simulink model "ADU_Integration_R2014a_simulation"  (R2014a)
settings: Solver=FixedStepDiscrete  StartTime=285  StopTime=300  FixedStep=0.01  RelTol=1e-3
PostLoadFcn:
  | , if any(exist('dsrtsu_mdlpostloadfcn', 'file') == [2, 3, 6]), try dsrtsu_mdlpostloadfcn('Execute', bdroot); catch fprintf('Error in PostLoadFcn (dsrtsu_mdlpostloadfcn) for model "%s":\n %s\n', bdroot, lasterr); end, end,
InitFcn:
  | load 'data/chi2_dat';
  | load 'data/Line_struct';
  | load 'data/innerLNM_1';
  | load 'data/middleLNM_2';
  | load 'data/outerLNM_1';
  | load 'data/landmarks_patac_schimmel_ccw';
  | load 'data/patac_navi_array';
  | load 'data/sensor';
  | load 'data/map_struct';
  | addpath map_src
  | Integration_Parameter;
  | load 'TestData_001';
values from neighbouring files (symbols this model uses):
  TestData_001 =     [TestData_001.mat]
undefined symbols (not defined in the file or in its folder): chi2_dat, innerLNM_1, landmarks_patac_schimmel_ccw, middleLNM_2, outerLNM_1, patac_navi_array
libraries: simulink x36, rtican x1
(part 13 of 22)

== stateflow chart ADU_Integration_R2014a_simulation/Fusion_Model/Fusion_Block/Side_Fusion/Side_Fusion ==
  state Gtj  = G_cal(xt,yt,xj,yj,P11,P12,P13,P14,P21,P22,P23,P24,... [function]
    P31,P32,P33,P34,P41,P42,P43,P44,R11,R12,R21,R22)
  state Set_Source(data) [function]
    (default) -> (junction 1307)
    (junction 1307) -> (junction 1308) : {
        | DataSource = data;
        | }
  state Tracker_Update [function]
    state Tracker_Filter [function]
      state Measurement_Select [function]
        state Data_Gen [function]
          (default) -> (junction 648)
          (junction 648) -> (junction 650) [order 1] : [j<Measure_Num]
          (junction 656) -> (junction 648) : {
              | j++;
              | }
          (junction 648) -> (junction 661) [order 2] : {
              | j=0;
              | }
          (junction 650) -> (junction 656) : {
              | P_Bulb[j][0]=Ptj[t][j];
              | P_Bulb[j][1]=Measure_Data[j][1]-FusDataInternal[t][1];
              | P_Bulb[j][2]=Measure_Data[j][2]-FusDataInternal[t][3];
              | P_Bulb[j][3]=j;%Used to define the measurement is used
              | }
        state Bulb_Sort [function]
          (default) -> (junction 638) : {
              | P_Bulbtemp0=0;P_Bulbtemp1=0;P_Bulbtemp2=0;
              | LoopFlg=1;
              | }
          (junction 2794) -> (junction 2793) [order 1] : [P_Bulb[j][0]>P_Bulb[j+1][0]]
          (junction 2800) -> (junction 2794) [order 1] : [j<Measure_Num-1]
          (junction 2813) -> (junction 2800) : {LoopFlg=0;}
          (junction 638) -> (junction 639) [order 1] : [LoopFlg==1]
          (junction 639) -> (junction 2813) [order 1] : [Measure_Num>2]
          (junction 2794) -> (junction 2790) [order 2]
          (junction 2793) -> (junction 2791) : {
              | P_Bulbtemp0=P_Bulb[j][0];P_Bulbtemp1=P_Bulb[j][1];
              | P_Bulbtemp2=P_Bulb[j][2];P_Bulbtemp3=P_Bulb[j][3];
              | P_Bulb[j][0]=P_Bulb[j+1][0];P_Bulb[j][1]=P_Bulb[j+1][1];
              | P_Bulb[j][2]=P_Bulb[j+1][2];P_Bulb[j][3]=P_Bulb[j+1][3];
              | P_Bulb[j+1][0]=P_Bulbtemp0;P_Bulb[j+1][1]=P_Bulbtemp1;
              | P_Bulb[j+1][2]=P_Bulbtemp2;P_Bulb[j+1][3]=P_Bulbtemp3;
              | LoopFlg=1;
              | }
          (junction 2817) -> (junction 638) : {
              | j=0;
              | }
          (junction 638) -> (junction 679) [order 2]
          (junction 2790) -> (junction 2800) : {
              | j++;
              | }
          (junction 2800) -> (junction 2802) [order 2]
          (junction 639) -> (junction 2815) [order 2]
          (junction 2815) -> (junction 2805) [order 1] : [Measure_Num>1]
          (junction 2805) -> (junction 2808) [order 1] : [P_Bulb[0][0]>P_Bulb[1][0]]
          (junction 2815) -> (junction 2817) [order 2] : {
              | LoopFlg=0;
              | }
          (junction 2805) -> (junction 675) [order 2] : {
              | LoopFlg=0;
              | }
          (junction 2808) -> (junction 2809) : {
              | P_Bulbtemp0=P_Bulb[0][0];P_Bulbtemp1=P_Bulb[0][1];
              | P_Bulbtemp2=P_Bulb[0][2];P_Bulbtemp3=P_Bulb[0][3];
              | P_Bulb[0][0]=P_Bulb[1][0];P_Bulb[0][1]=P_Bulb[1][1];
              | P_Bulb[0][2]=P_Bulb[1][2];P_Bulb[0][3]=P_Bulb[1][3];
              | P_Bulb[1][0]=P_Bulbtemp0;P_Bulb[1][1]=P_Bulbtemp1;
              | P_Bulb[1][2]=P_Bulbtemp2;P_Bulb[1][3]=P_Bulbtemp3;
              | LoopFlg=0;
              | }
          (junction 2791) -> (junction 2790)
          (junction 675) -> (junction 2817)
          (junction 2802) -> (junction 2809)
          (junction 2809) -> (junction 675)
        state Measure_Select [function]
          note: this part is select the 6  highest possible measurement to update
              | Tracker, and make sure if possible lower than 15%, think the date
              | as unused.
          (default) -> (junction 682) : {mk=0;}
          (junction 682) -> (junction 2830) [order 1] : [Measure_Num>2]
          (junction 2830) -> (junction 2829) [order 1] : [k<3]
          (junction 2829) -> (junction 2825) [order 1] : [P_Bulb[Measure_Num-1-k][0]>Poss_Threshold_used]
          (junction 2826) -> (junction 2830) : {
              | k++;
              | }
          (junction 682) -> (junction 715) [order 2]
          (junction 2830) -> (junction 2832) [order 2]
          (junction 2829) -> (junction 2826) [order 2]
          (junction 2825) -> (junction 2821) : {
              | SelectMea[k][0]=P_Bulb[Measure_Num-1-k][0];
              | SelectMea[k][1]=P_Bulb[Measure_Num-1-k][1];
              | SelectMea[k][2]=P_Bulb[Measure_Num-1-k][2];
              | Measure_Data[P_Bulb[Measure_Num-1-k][3]][4]=1;%Means that the measurement is used
              | mk++;
              | }
          (junction 2832) -> (junction 715)
          (junction 2821) -> (junction 2826)
          (junction 715) -> (junction 2835) : {
              | k=0;
              | }
          (junction 2837) -> (junction 2849) [order 1] : [k<2]
          (junction 2835) -> (junction 2837) [order 1] : [Measure_Num==2]
          (junction 2849) -> (junction 2847) [order 1] : [P_Bulb[Measure_Num-1-k][0]>Poss_Threshold_used]
          (junction 2844) -> (junction 2837) : {
              | k++;
              | }
          (junction 2849) -> (junction 2844) [order 2]
          (junction 2835) -> (junction 2853) [order 2]
          (junction 2837) -> (junction 2850) [order 2]
          (junction 2847) -> (junction 2846) : {
              | SelectMea[k][0]=P_Bulb[Measure_Num-1-k][0];
              | SelectMea[k][1]=P_Bulb[Measure_Num-1-k][1];
              | SelectMea[k][2]=P_Bulb[Measure_Num-1-k][2];
              | Measure_Data[P_Bulb[Measure_Num-1-k][3]][4]=1;%Means that the measurement is used
              | mk++;
              | }
          (junction 2850) -> (junction 2853)
          (junction 2846) -> (junction 2844)
          (junction 2853) -> (junction 2871) : {
              | k=0;
              | }
          (junction 2867) -> (junction 2861) [order 1] : [k<1]
          (junction 2871) -> (junction 2867) [order 1] : [Measure_Num==1]
          (junction 2861) -> (junction 2872) [order 1] : [P_Bulb[Measure_Num-1-k][0]>Poss_Threshold_used]
          (junction 2868) -> (junction 2867) : {
              | k++;
              | }
          (junction 2861) -> (junction 2868) [order 2]
          (junction 2871) -> (junction 2873) [order 2]
          (junction 2867) -> (junction 2865) [order 2]
          (junction 2872) -> (junction 2866) : {
              | SelectMea[k][0]=P_Bulb[Measure_Num-1-k][0];
              | SelectMea[k][1]=P_Bulb[Measure_Num-1-k][1];
              | SelectMea[k][2]=P_Bulb[Measure_Num-1-k][2];
              | Measure_Data[P_Bulb[Measure_Num-1-k][3]][4]=1;%Means that the measurement is used
              | mk++;
              | }
          (junction 2865) -> (junction 2873)
          (junction 2866) -> (junction 2868)
          (junction 2873) -> (junction 2875) : {
              | k=0;
              | }
          (junction 2875) -> (junction 3173)
          (junction 3173) -> (junction 3175) [order 1] : [mk==1]%means that the tracker
              | %only has one measurement
          (junction 3175) -> (junction 3177) [order 1] : [OneMeasureFlg[P_Bulb[Measure_Num-1-k][3]]==1]
              | %Means that the measurement has used for another tracker
              | %and this tracker only has one measurement
          (junction 3173) -> (junction 3184) [order 2]
          (junction 3175) -> (junction 3181) [order 2] : {
              | OneMeasureFlg[P_Bulb[Measure_Num-1-k][3]]=1;
              | %Means that this measurement has used for another track and the track
              | %only has one measurement
              | }
          (junction 3177) -> (junction 3179) : {
              | mk=0;%Means that no measurement here
              | }
          (junction 3181) -> (junction 3184)
          (junction 3179) -> (junction 3181)
          (junction 3184) -> (junction 3187)
          (junction 3187) -> (junction 3280) [order 1] : [j<Measure_Num]
          (junction 3280) -> (junction 3282) [order 1] : [P_Bulb[j][0]>Poss_Threshold_unused]
          (junction 3286) -> (junction 3187) : {
              | j++;
              | }
          (junction 3187) -> (junction 3290) [order 2] : {
              | j=0;
              | }
          (junction 3280) -> (junction 3286) [order 2]
          (junction 3282) -> (junction 3284) : {
              | Measure_Data[P_Bulb[j][3]][4]=1;
              | }
          (junction 3284) -> (junction 3286)
        (default) -> (junction 630) : {
            | LoopFlg=1;SelectMea=0;
            | %This Step is to select measurements to update the tracker, the measurement used
            | }
        (junction 630) -> (junction 635) : {
            | Data_Gen();
            | Bulb_Sort();
            | Measure_Select();
            | }
      state Update [function]
        state [RangeX,VelX,RangeY,VelY,P11,P12,P13,P14,P21,P22,P23,P24,P31,P32,P33,P34,P41,P42,P43,... [function]
          P44] = Update(Pre_x,Pre_vx,Pre_y,Pre_vy,pre_p11,pre_p12,pre_p13,pre_p14,pre_p21,pre_p22,...
          pre_p23,pre_p24,pre_p31,pre_p32,pre_p33,pre_p34,pre_p41,pre_p42,pre_p43,pre_p44,mk,m00,...
          m01,m2,m10,m11,m12,m20,m21,m22,Pt0)
        (default) -> (junction 718)
        (junction 718) -> (junction 768) [order 1] : [mk>0]%Exist Measurement can update Tracker
        (junction 718) -> (junction 719) [order 2] : {
            | UpdateTrackFlag[t]=0;%Could not find measurement to update tracker
            | FusDataInternal_temp[t][0]=FusDataInternal[t][0];FusDataInternal_temp[t][1]=FusDataInternal[t][1];
            | FusDataInternal_temp[t][2]=FusDataInternal[t][2];FusDataInternal_temp[t][3]=FusDataInternal[t][3];
            | FusDataInternal_temp[t][4]=FusDataInternal[t][4];FusDataInternal_temp[t][5]=FusDataInternal[t][5];
            | FusDataInternal_temp[t][6]=FusDataInternal[t][6];FusDataInternal_temp[t][7]=FusDataInternal[t][7];
            | FusDataInternal_temp[t][8]=FusDataInternal[t][8];FusDataInternal_temp[t][9]=FusDataInternal[t][9];
            | FusDataInternal_temp[t][10]=FusDataInternal[t][10];FusDataInternal_temp[t][11]=FusDataInternal[t][11];
            | FusDataInternal_temp[t][12]=FusDataInternal[t][12];FusDataInternal_temp[t][13]=FusDataInternal[t][13];
            | FusDataInternal_temp[t][14]=FusDataInternal[t][14];FusDataInternal_temp[t][15]=FusDataInternal[t][15];
            | FusDataInternal_temp[t][16]=FusDataInternal[t][16];FusDataInternal_temp[t][17]=FusDataInternal[t][17];
            | FusDataInternal_temp[t][18]=FusDataInternal[t][18];FusDataInternal_temp[t][19]=FusDataInternal[t][19];
            | FusDataInternal_temp[t][20]=FusDataInternal[t][20];FusDataInternal_temp[t][21]=FusDataInternal[t][21];
            | FusDataInternal_temp[t][22]=FusDataInternal[t][22];
            | FusDataInternal_temp[t][23]=FusDataInternal[t][23];FusDataInternal_temp[t][24]=FusDataInternal[t][24];
            | }
        (junction 768) -> (junction 771) : {
            | UpdateTrackFlag[t]=1;
            | [FusDataInternal_temp[t][1],FusDataInternal_temp[t][2],FusDataInternal_temp[t][3],FusDataInternal_temp[t][4],...
            | FusDataInternal_temp[t][7],FusDataInternal_temp[t][8],FusDataInternal_temp[t][9],FusDataInternal_temp[t][10],...
            | FusDataInternal_temp[t][11],FusDataInternal_temp[t][12],FusDataInternal_temp[t][13],FusDataInternal_temp[t][14],...
            | FusDataInternal_temp[t][15],FusDataInternal_temp[t][16],FusDataInternal_temp[t][17],FusDataInternal_temp[t][18],...
            | FusDataInternal_temp[t][19],FusDataInternal_temp[t][20],FusDataInternal_temp[t][21],FusDataInternal_temp[t][22]]=Update(FusDataInternal[t][1],...
            | FusDataInternal[t][2],FusDataInternal[t][3],FusDataInternal[t][4],FusDataInternal[t][7],FusDataInternal[t][8],FusDataInternal[t][9],...
            | FusDataInternal[t][10],FusDataInternal[t][11],FusDataInternal[t][12],FusDataInternal[t][13],FusDataInternal[t][14],FusDataInternal[t][15],...
            | FusDataInternal[t][16],FusDataInternal[t][17],FusDataInternal[t][18],FusDataInternal[t][19],FusDataInternal[t][20],FusDataInternal[t][21],...
            | FusDataInternal[t][22],mk,SelectMea[0][0],SelectMea[0][1],SelectMea[0][2],SelectMea[1][0],SelectMea[1][1],SelectMea[1][2],SelectMea[2][0],...
            | SelectMea[2][1],SelectMea[2][2],(1-Ptsum[t]));
            | FusDataInternal_temp[t][0]=FusDataInternal[t][0];FusDataInternal_temp[t][5]=FusDataInternal[t][5];FusDataInternal_temp[t][6]=FusDataInternal[t][6];
            | FusDataInternal_temp[t][23]=FusDataInternal[t][23];FusDataInternal_temp[t][24]=FusDataInternal[t][24];
            | }
        (junction 771) -> (junction 719)
        (junction 719) -> (junction 825)
      (default) -> (junction 626)
      (junction 626) -> (junction 627) : {
          | Measurement_Select();
          | Update();
          | }
    (default) -> (junction 607)
    (junction 607) -> (junction 608) [order 1] : [t<Num_Trg]
    (junction 610) -> (junction 607) : {
        | t++;
        | }
    (junction 607) -> (junction 613) [order 2] : {
        | t=0;
        | }
    (junction 608) -> (junction 610) : {
        | Tracker_Filter();
        | }
  state Set_Time(data) [function]
    (default) -> (junction 1301)
    (junction 1301) -> (junction 1302) : {
        | Sensor_sampleTime = data;
        | }
  state FusDataIni [function]
    (default) -> (junction 206)
    (junction 206) -> (junction 207) : {
        | %deltaT=0;
        | deltaT=Sensor_sampleTime-LastCalTime;
        | TrackCounter=0;c=0;Num_Out=0;
        | Gtj=0;Ptj=0;Measure_Data=0;Gtsum=0;Gsumj=0;Ptsum=0;Psumj=0;
        | Measure_Data=0;Measure_Num=0;Tracker_Num=0;k=0;n=0;t=0;j=0;
        | SideFusOut=0;Returns=0;Num_Returns=0;OneMeasureFlg=0;
        | FusDataInternal=0;Pt0=0;P_Bulb=0;UpdateTrackFlag=0;SelectMea=0;
        | }
    (junction 207) -> (junction 208)
  state FusTrackPredict [function]
    state [RangeX,VelX,RangeY,VelY,P11,P12,P13,P14,P21,P22,P23,P24,P31,P32,P33,P34,P41,P42,P43,... [function]
      P44] = Forecast(Pre_x,Pre_vx,Pre_y,Pre_vy,deltaT,pre_p11,pre_p12,pre_p13,pre_p14,pre_p21,...
      pre_p22,pre_p23,pre_p24,pre_p31,pre_p32,pre_p33,pre_p34,pre_p41,pre_p42,pre_p43,pre_p44)
    (default) -> (junction 330)
    (junction 330) -> (junction 331) [order 1] : [k<Num_Trg]
    (junction 331) -> (junction 332) [order 1] : [FusDataInternal_temp[k][0]!=0]
    (junction 333) -> (junction 330) : {
        | k++;
        | }
    (junction 330) -> (junction 335) [order 2] : {
        | Num_Trg=n;
        | n=0;
        | }
    (junction 331) -> (junction 333) [order 2]
    (junction 332) -> (junction 334) : {
        | [FusDataInternal[n][1],FusDataInternal[n][2],FusDataInternal[n][3],FusDataInternal[n][4],FusDataInternal[n][7],FusDataInternal[n][8],FusDataInternal[n][9],FusDataInternal[n][10],...
        | FusDataInternal[n][11],FusDataInternal[n][12],FusDataInternal[n][13],FusDataInternal[k][14],FusDataInternal[k][15],FusDataInternal[k][16],FusDataInternal[n][17],FusDataInternal[n][18],...
        | FusDataInternal[n][19],FusDataInternal[n][20],FusDataInternal[n][21],FusDataInternal[n][22]]=Forecast(FusDataInternal_temp[k][1],FusDataInternal_temp[k][2],FusDataInternal_temp[k][3],...
        | FusDataInternal_temp[k][4],deltaT,FusDataInternal_temp[k][7],FusDataInternal_temp[k][8],FusDataInternal_temp[k][9],FusDataInternal_temp[k][10],FusDataInternal_temp[k][11],FusDataInternal_temp[k][12],...
        | FusDataInternal_temp[k][13],FusDataInternal_temp[k][14],FusDataInternal_temp[k][15],FusDataInternal_temp[k][16],FusDataInternal_temp[k][17],FusDataInternal_temp[k][18],FusDataInternal_temp[k][19],...
        | FusDataInternal_temp[k][20],FusDataInternal_temp[k][21],FusDataInternal_temp[k][22]);%All fusion targets forecast,after this step, target number in FusDataInternal is the same as last calculation, but forecast with delta time
        | FusDataInternal[n][0]=FusDataInternal_temp[k][0];FusDataInternal[n][5]=FusDataInternal_temp[k][5];FusDataInternal[n][6]=FusDataInternal_temp[k][6];
        | FusDataInternal[n][23]=FusDataInternal_temp[k][23];FusDataInternal[n][24]=FusDataInternal_temp[k][24];
        | n++;
        | }
    (junction 334) -> (junction 333)
  state Tracker_Initial [function]
    state Unused_Return_Gen [function]
      (default) -> (junction 1656) : {
          | Num_Returns=0;
          | }
      (junction 1656) -> (junction 1662) [order 1] : [k<Measure_Num]
      (junction 1662) -> (junction 1664) [order 1] : [Measure_Data[k][4]==0]
      (junction 1670) -> (junction 1656) : {
          | k++;
          | }
      (junction 1656) -> (junction 1674) [order 2] : {
          | k=0;
          | }
      (junction 1662) -> (junction 1670) [order 2]
      (junction 1664) -> (junction 1666) : {
          | Returns[Num_Returns][0]=Measure_Data[k][1];
          | Returns[Num_Returns][1]=Measure_Data[k][2];
          | Returns[Num_Returns][2]=Measure_Data[k][4];
          | Num_Returns++;
          | }
      (junction 1666) -> (junction 1670)
    state LFSRR_Ini [function]
      state LFSRR_Ini_Update [function]
        note: %Recently used in 4/5 logical modle in the initial of radar tracker
        state Ini_FifthTime_LF [function]
          (default) -> (junction 2080) : {
              | RelDeg=0;Min_Distance_IniTrack=9;RelativeDist=0;
              | x_5_predict=3*Ini_Tracker_LFSRR[k][10]-3*Ini_Tracker_LFSRR[k][8]+Ini_Tracker_LFSRR[k][6];%Use three point to predict next point based constant acc
              | y_5_predict=3*Ini_Tracker_LFSRR[k][11]-3*Ini_Tracker_LFSRR[k][9]+Ini_Tracker_LFSRR[k][7];%Use three point to predict next point based constant acc
              | Updatereturn=0;Ini_Tracker_UpdateFlg=0;
              | }
          (junction 2080) -> (junction 2890) [order 1] : [(j<Num_Returns)]
          (junction 2890) -> (junction 2091) [order 1] : [(Returns[j][2]==0)]
          (junction 2892) -> (junction 2080) : {
              | j++;
              | }
          (junction 2091) -> (junction 2108) : {
              | RelativeDist=(x_5_predict-Returns[j][0])*(x_5_predict-Returns[j][0])+(y_5_predict-Returns[j][1])*(y_5_predict-Returns[j][1]);
              | RelDeg=cos_cal(Ini_Tracker_LFSRR[k][8],Ini_Tracker_LFSRR[k][9],...
              | Ini_Tracker_LFSRR[k][10],Ini_Tracker_LFSRR[k][11],Returns[j][0],Returns[j][1]);
              | }
          (junction 2080) -> (junction 2102) [order 2] : {
              | j=0;
              | }
          (junction 2890) -> (junction 2892) [order 2]
          (junction 2108) -> (junction 2987) [order 1] : [(RelativeDist<4)]
          (junction 2987) -> (junction 2990) [order 1] : [(RelativeDist<0.1)]
          (junction 2108) -> (junction 2107) [order 2]
          (junction 2987) -> (junction 2991) [order 2]
          (junction 2990) -> (junction 2973)
          (junction 2991) -> (junction 2973) [order 1] : [(((RelDeg>120) || (RelDeg<60)))]
          (junction 2973) -> (junction 2977) [order 1] : [RelativeDist<Min_Distance_IniTrack]
          (junction 2991) -> (junction 2985) [order 2]
          (junction 2973) -> (junction 2981) [order 2]
          (junction 2977) -> (junction 2979) : {
              | Updatereturn=j;
              | Ini_Tracker_UpdateFlg=1;
              | Min_Distance_IniTrack=RelativeDist;
              | }
          (junction 2981) -> (junction 2985)
          (junction 2979) -> (junction 2981)
          (junction 2985) -> (junction 2107)
          (junction 2107) -> (junction 2892)
          (junction 2102) -> (junction 2104) [order 1] : [Ini_Tracker_UpdateFlg==1]%Means that the tracker k found measurement
          (junction 2102) -> (junction 2094) [order 2] : {
              | %cound not found, and enter 5 searches means that could not found once before, so delete
              | }
          (junction 2104) -> (junction 2100) : {
              | Returns[Updatereturn][2]=1;
              | %Which means that the return is used
              | TrackIni(Returns[Updatereturn][0],Returns[Updatereturn][1]);
              | }
          (junction 2100) -> (junction 2094)
          (junction 2094) -> (junction 2105) : {
              | Updatereturn=0;Ini_Tracker_UpdateFlg=0;
              | }
        state Ini_ForthTime_LF [function]
          (default) -> (junction 2039) : {
              | RelDeg=0;Min_Distance_IniTrack=9;RelativeDist=0;
              | x_4_predict=3*Ini_Tracker_LFSRR[k][8]-3*Ini_Tracker_LFSRR[k][6]+Ini_Tracker_LFSRR[k][4];%Use three point to predict next point based constant acc
              | y_4_predict=3*Ini_Tracker_LFSRR[k][9]-3*Ini_Tracker_LFSRR[k][7]+Ini_Tracker_LFSRR[k][5];%Use three point to predict next point based constant acc
              | Updatereturn=0;Ini_Tracker_UpdateFlg=0;
              | }
          (junction 2039) -> (junction 2885) [order 1] : [(j<Num_Returns)]
          (junction 2885) -> (junction 2047) [order 1] : [(Returns[j][2]==0)]
          (junction 2887) -> (junction 2039) : {
              | j++;
              | }
          (junction 2047) -> (junction 2044) : {
              | RelativeDist=(x_4_predict-Returns[j][0])*(x_4_predict-Returns[j][0])+(y_4_predict-Returns[j][1])*(y_4_predict-Returns[j][1]);
              | RelDeg=cos_cal(Ini_Tracker_LFSRR[k][6],Ini_Tracker_LFSRR[k][7],...
              | Ini_Tracker_LFSRR[k][8],Ini_Tracker_LFSRR[k][9],Returns[j][0],Returns[j][1]);
              | }
          (junction 2039) -> (junction 2053) [order 2] : {
              | j=0;
              | }
          (junction 2885) -> (junction 2887) [order 2]
          (junction 2044) -> (junction 2967) [order 1] : [(RelativeDist<4)]
          (junction 2967) -> (junction 2970) [order 1] : [(RelativeDist<0.1)]
          (junction 2044) -> (junction 2036) [order 2]
          (junction 2967) -> (junction 2971) [order 2]
          (junction 2970) -> (junction 2953)
          (junction 2971) -> (junction 2953) [order 1] : [(((RelDeg>120) || (RelDeg<60)))]
          (junction 2953) -> (junction 2957) [order 1] : [RelativeDist<Min_Distance_IniTrack]
          (junction 2971) -> (junction 2965) [order 2]
          (junction 2953) -> (junction 2961) [order 2]
          (junction 2957) -> (junction 2959) : {
              | Updatereturn=j;
              | Ini_Tracker_UpdateFlg=1;
              | Min_Distance_IniTrack=RelativeDist;
              | }
          (junction 2036) -> (junction 2887)
          (junction 2965) -> (junction 2036)
          (junction 2961) -> (junction 2965)
          (junction 2959) -> (junction 2961)
          (junction 2053) -> (junction 2052) [order 1] : [Ini_Tracker_UpdateFlg==1]%Means that the tracker k found measurement
          (junction 2052) -> (junction 2064) [order 1] : [Ini_Tracker_LFSRR[k][3]==3]%Has found measurement 4 times and begin ini
          (junction 2053) -> (junction 2071) [order 2]
          (junction 2052) -> (junction 2049) [order 2] : {
              | Returns[Updatereturn][2]=1;%Which means that the return is used
              | Ini_Tracker_LFSRR_New[Num_Ini_Tracker_LFSRR_New][0]=Returns[Updatereturn][0];
              | Ini_Tracker_LFSRR_New[Num_Ini_Tracker_LFSRR_New][1]=Returns[Updatereturn][1];
              | Ini_Tracker_LFSRR_New[Num_Ini_Tracker_LFSRR_New][2]=4;%Tracker counter
              | Ini_Tracker_LFSRR_New[Num_Ini_Tracker_LFSRR_New][3]=3;%Association counter
              | Ini_Tracker_LFSRR_New[Num_Ini_Tracker_LFSRR_New][4]=Ini_Tracker_LFSRR[k][4];
              | Ini_Tracker_LFSRR_New[Num_Ini_Tracker_LFSRR_New][5]=Ini_Tracker_LFSRR[k][5];
              | Ini_Tracker_LFSRR_New[Num_Ini_Tracker_LFSRR_New][6]=Ini_Tracker_LFSRR[k][6];
              | Ini_Tracker_LFSRR_New[Num_Ini_Tracker_LFSRR_New][7]=Ini_Tracker_LFSRR[k][7];
              | Ini_Tracker_LFSRR_New[Num_Ini_Tracker_LFSRR_New][8]=Ini_Tracker_LFSRR[k][8];
              | Ini_Tracker_LFSRR_New[Num_Ini_Tracker_LFSRR_New][9]=Ini_Tracker_LFSRR[k][9];
              | Ini_Tracker_LFSRR_New[Num_Ini_Tracker_LFSRR_New][10]=Returns[Updatereturn][0];
              | Ini_Tracker_LFSRR_New[Num_Ini_Tracker_LFSRR_New][11]=Returns[Updatereturn][1];
              | Num_Ini_Tracker_LFSRR_New++;
              | }
          (junction 2064) -> (junction 2068) : {
              | Returns[Updatereturn][2]=1;
              | %Which means that the return is used
              | TrackIni(Returns[Updatereturn][0],Returns[Updatereturn][1]);
              | }
          (junction 2071) -> (junction 2073) [order 1] : [Ini_Tracker_LFSRR[k][3]==3]
              | %Has found measurement 3 times before
          (junction 2073) -> (junction 2075) : {
              | Ini_Tracker_LFSRR_New[Num_Ini_Tracker_LFSRR_New][0]=x_4_predict;
              | Ini_Tracker_LFSRR_New[Num_Ini_Tracker_LFSRR_New][1]=y_4_predict;
              | Ini_Tracker_LFSRR_New[Num_Ini_Tracker_LFSRR_New][2]=4;%Tracker counter
              | Ini_Tracker_LFSRR_New[Num_Ini_Tracker_LFSRR_New][3]=3;%Association counter
              | Ini_Tracker_LFSRR_New[Num_Ini_Tracker_LFSRR_New][4]=Ini_Tracker_LFSRR[k][4];
              | Ini_Tracker_LFSRR_New[Num_Ini_Tracker_LFSRR_New][5]=Ini_Tracker_LFSRR[k][5];
              | Ini_Tracker_LFSRR_New[Num_Ini_Tracker_LFSRR_New][6]=Ini_Tracker_LFSRR[k][6];
              | Ini_Tracker_LFSRR_New[Num_Ini_Tracker_LFSRR_New][7]=Ini_Tracker_LFSRR[k][7];
              | Ini_Tracker_LFSRR_New[Num_Ini_Tracker_LFSRR_New][8]=Ini_Tracker_LFSRR[k][8];
              | Ini_Tracker_LFSRR_New[Num_Ini_Tracker_LFSRR_New][9]=Ini_Tracker_LFSRR[k][9];
              | Ini_Tracker_LFSRR_New[Num_Ini_Tracker_LFSRR_New][10]=x_4_predict;
              | Ini_Tracker_LFSRR_New[Num_Ini_Tracker_LFSRR_New][11]=y_4_predict;
              | Num_Ini_Tracker_LFSRR_New++;
              | }
          (junction 2071) -> (junction 2054) [order 2] : {
              | %Cound not found measurement twice,
              | % So not transfer tracker k to new list
              | }
          (junction 2075) -> (junction 2054)
          (junction 2049) -> (junction 2075)
          (junction 2068) -> (junction 2049)
          (junction 2054) -> (junction 2057) : {
              | Updatereturn=0;Ini_Tracker_UpdateFlg=0;
              | }
        state Ini_ThridTime_LF [function]
          (default) -> (junction 1976) : {
              | RelDeg=0;Min_Distance_IniTrack=9;RelativeDist=0;
              | x_3_predict=2*Ini_Tracker_LFSRR[k][6]-Ini_Tracker_LFSRR[k][4];%Use two point to predict next point based constant velocity
              | y_3_predict=2*Ini_Tracker_LFSRR[k][7]-Ini_Tracker_LFSRR[k][5];%Use two point to predict next point based constant velocity
              | Updatereturn=0;Ini_Tracker_UpdateFlg=0;
              | }
          (junction 1976) -> (junction 2878) [order 1] : [(j<Num_Returns)]
          (junction 2878) -> (junction 1977) [order 1] : [(Returns[j][2]==0)]
          (junction 2882) -> (junction 1976) : {
              | j++;
              | }
          (junction 1977) -> (junction 1978) : {
              | RelativeDist=(x_3_predict-Returns[j][0])*(x_3_predict-Returns[j][0])+(y_3_predict-Returns[j][1])*(y_3_predict-Returns[j][1]);
              | RelDeg=cos_cal(Ini_Tracker_LFSRR[k][4],Ini_Tracker_LFSRR[k][5],...
              | Ini_Tracker_LFSRR[k][6],Ini_Tracker_LFSRR[k][7],Returns[j][0],Returns[j][1]);
              | }
          (junction 1976) -> (junction 2024) [order 2] : {
              | j=0;
              | }
          (junction 2878) -> (junction 2882) [order 2]
          (junction 2942) -> (junction 2946) [order 1] : [(RelativeDist<0.1)]
          (junction 1978) -> (junction 2942) [order 1] : [(RelativeDist<4)]
          (junction 1978) -> (junction 2003) [order 2]
          (junction 2942) -> (junction 2944) [order 2]
          (junction 2946) -> (junction 2001)
          (junction 2944) -> (junction 2001) [order 1] : [(((RelDeg>120) || (RelDeg<60)))]
          (junction 2001) -> (junction 2013) [order 1] : [RelativeDist<Min_Distance_IniTrack]
          (junction 2944) -> (junction 2949) [order 2]
          (junction 2001) -> (junction 2020) [order 2]
          (junction 2013) -> (junction 2018) : {
              | Updatereturn=j;
              | Ini_Tracker_UpdateFlg=1;
              | Min_Distance_IniTrack=RelativeDist;
              | }
          (junction 2003) -> (junction 2882)
          (junction 2949) -> (junction 2003)
          (junction 2020) -> (junction 2949)
          (junction 2018) -> (junction 2020)
          (junction 2024) -> (junction 2025) [order 1] : [Ini_Tracker_UpdateFlg==1]%Means that the tracker k found measurement
          (junction 2024) -> (junction 2029) [order 2] : {
              | Ini_Tracker_LFSRR_New[Num_Ini_Tracker_LFSRR_New][0]=x_3_predict;
              | Ini_Tracker_LFSRR_New[Num_Ini_Tracker_LFSRR_New][1]=y_3_predict;
              | Ini_Tracker_LFSRR_New[Num_Ini_Tracker_LFSRR_New][2]=3;%Tracker counter
              | Ini_Tracker_LFSRR_New[Num_Ini_Tracker_LFSRR_New][3]=2;%Association counter
              | Ini_Tracker_LFSRR_New[Num_Ini_Tracker_LFSRR_New][4]=Ini_Tracker_LFSRR[k][4];
              | Ini_Tracker_LFSRR_New[Num_Ini_Tracker_LFSRR_New][5]=Ini_Tracker_LFSRR[k][5];
              | Ini_Tracker_LFSRR_New[Num_Ini_Tracker_LFSRR_New][6]=Ini_Tracker_LFSRR[k][6];
              | Ini_Tracker_LFSRR_New[Num_Ini_Tracker_LFSRR_New][7]=Ini_Tracker_LFSRR[k][7];
              | Ini_Tracker_LFSRR_New[Num_Ini_Tracker_LFSRR_New][8]=x_3_predict;
              | Ini_Tracker_LFSRR_New[Num_Ini_Tracker_LFSRR_New][9]=y_3_predict;
              | Num_Ini_Tracker_LFSRR_New++;
              | }
          (junction 2025) -> (junction 2027) : {
              | Returns[Updatereturn][2]=1;%Which means that the return is used
              | Ini_Tracker_LFSRR_New[Num_Ini_Tracker_LFSRR_New][0]=Returns[Updatereturn][0];
              | Ini_Tracker_LFSRR_New[Num_Ini_Tracker_LFSRR_New][1]=Returns[Updatereturn][1];
              | Ini_Tracker_LFSRR_New[Num_Ini_Tracker_LFSRR_New][2]=3;%Tracker counter
              | Ini_Tracker_LFSRR_New[Num_Ini_Tracker_LFSRR_New][3]=3;%Association counter
              | Ini_Tracker_LFSRR_New[Num_Ini_Tracker_LFSRR_New][4]=Ini_Tracker_LFSRR[k][4];
              | Ini_Tracker_LFSRR_New[Num_Ini_Tracker_LFSRR_New][5]=Ini_Tracker_LFSRR[k][5];
              | Ini_Tracker_LFSRR_New[Num_Ini_Tracker_LFSRR_New][6]=Ini_Tracker_LFSRR[k][6];
              | Ini_Tracker_LFSRR_New[Num_Ini_Tracker_LFSRR_New][7]=Ini_Tracker_LFSRR[k][7];
              | Ini_Tracker_LFSRR_New[Num_Ini_Tracker_LFSRR_New][8]=Returns[Updatereturn][0];
              | Ini_Tracker_LFSRR_New[Num_Ini_Tracker_LFSRR_New][9]=Returns[Updatereturn][1];
              | Num_Ini_Tracker_LFSRR_New++;
              | }
          (junction 2027) -> (junction 2029)
          (junction 2029) -> (junction 2032) : {
              | Updatereturn=0;Ini_Tracker_UpdateFlg=0;
              | }
        state Ini_SecondTime_LF [function]
          (default) -> (junction 1821) : {
              | AssoFlgtm=0;
              | }
          (junction 1821) -> (junction 1894) [order 1] : [j<Num_Returns]
          (junction 1896) -> (junction 1821) : {
              | j++;
              | }
          (junction 1821) -> (junction 1934) [order 2] : {
              | j=0;
              | }
          (junction 1894) -> (junction 1896) : {
              | AssoFlgtm[j]=VelocityMethod(Ini_Tracker_LFSRR[k][4],Ini_Tracker_LFSRR[k][5],...
              | Returns[j][0],Returns[j][1],10,1,5,0,1.5,1.5,9,0.04);%Velocity Association method
              | }
          (junction 1934) -> (junction 1936) [order 1] : [j<Num_Returns]
          (junction 1936) -> (junction 1938) [order 1] : [AssoFlgtm[j]==1]
          (junction 1940) -> (junction 1934) : {
              | j++;
              | }
          (junction 1934) -> (junction 1974) [order 2] : {
              | j=0;
              | AssoFlgtm=0;
              | }
          (junction 1936) -> (junction 1940) [order 2]
          (junction 1938) -> (junction 1943) : {
              | Returns[j][2]=1;%Which means that the return is used
              | Ini_Tracker_LFSRR_New[Num_Ini_Tracker_LFSRR_New][0]=Returns[j][0];
              | Ini_Tracker_LFSRR_New[Num_Ini_Tracker_LFSRR_New][1]=Returns[j][1];
              | Ini_Tracker_LFSRR_New[Num_Ini_Tracker_LFSRR_New][2]=2;
              | Ini_Tracker_LFSRR_New[Num_Ini_Tracker_LFSRR_New][3]=2;
              | Ini_Tracker_LFSRR_New[Num_Ini_Tracker_LFSRR_New][4]=Ini_Tracker_LFSRR[k][4];
              | Ini_Tracker_LFSRR_New[Num_Ini_Tracker_LFSRR_New][5]=Ini_Tracker_LFSRR[k][5];
              | Ini_Tracker_LFSRR_New[Num_Ini_Tracker_LFSRR_New][6]=Returns[j][0];
              | Ini_Tracker_LFSRR_New[Num_Ini_Tracker_LFSRR_New][7]=Returns[j][1];
              | Num_Ini_Tracker_LFSRR_New++;
              | }
          (junction 1943) -> (junction 1940)
        (default) -> (junction 1747)
        (junction 1747) -> (junction 1750) [order 1] : [Ini_Tracker_LFSRR[k][2]==4]%This Tracker has updated forth and find fifth measurement
        (junction 1747) -> (junction 1764) [order 2]
        (junction 1750) -> (junction 1762) : {
            | Ini_FifthTime_LF();
            | }
        (junction 1762) -> (junction 1764)
        (junction 1764) -> (junction 1772)
        (junction 1772) -> (junction 1774) [order 1] : [Ini_Tracker_LFSRR[k][2]==3]%This Tracker has updated thrid and find forth measurement
        (junction 1772) -> (junction 1770) [order 2]
        (junction 1774) -> (junction 1771) : {
            | Ini_ForthTime_LF();
            | }
        (junction 1771) -> (junction 1770)
        (junction 1770) -> (junction 1778)
        (junction 1778) -> (junction 1780) [order 1] : [Ini_Tracker_LFSRR[k][2]==2]%This Tracker has updated once and find thrid measurement
        (junction 1778) -> (junction 1783) [order 2]
        (junction 1780) -> (junction 1779) : {
            | Ini_ThridTime_LF();
            | }
        (junction 1779) -> (junction 1783)
        (junction 1783) -> (junction 1966)
        (junction 1966) -> (junction 1964) [order 1] : [Ini_Tracker_LFSRR[k][2]==1]%This Tracker is first initial and use velocity to find next measurements
        (junction 1966) -> (junction 1967) [order 2]
        (junction 1964) -> (junction 1965) : {
            | Ini_SecondTime_LF();
            | }
        (junction 1965) -> (junction 1967)
        (junction 1967) -> (junction 1969)
      state LFFirstTrackGen [function]
        (default) -> (junction 3322)
        (junction 3322) -> (junction 3324) [order 1] : [Num_Returns>1]%Two return, begine compare
        (junction 3322) -> (junction 3356) [order 2]
        (junction 3324) -> (junction 3304) : {
            | j=1;
            | }
        (junction 3318) -> (junction 3316) [order 1] : [(Returns[k][0]-Returns[j][0])*(Returns[k][0]-Returns[j][0])+...
            | (Returns[k][1]-Returns[j][1])*(Returns[k][1]-Returns[j][1])<=9]
        (junction 3309) -> (junction 3318) [order 1] : [Returns[j][2]==0]
        (junction 3297) -> (junction 3299) [order 1] : [Returns[k][2]==0]
        (junction 3299) -> (junction 3309) [order 1] : [j<Num_Returns]
        (junction 3304) -> (junction 3297) [order 1] : [k<Num_Returns-1]
        (junction 3311) -> (junction 3299) : {
            | j++;
            | }
        (junction 3318) -> (junction 3330) [order 2]
        (junction 3316) -> (junction 3328) : {
            | Group_Data[Group_Num][0]=Returns[j][0];
            | Group_Data[Group_Num][1]=Returns[j][1];
            | Returns[j][2]=1;
            | Group_Num=Group_Num+1;
            | }
        (junction 3303) -> (junction 3304) : {
            | k++;
            | j=k+1;
            | Group_Num=0;
            | Group_Data=0;
            | Group_X=0;
            | Group_Y=0;
            | }
        (junction 3297) -> (junction 3303) [order 2]
        (junction 3299) -> (junction 3314) [order 2] : {
            | Group_X=Returns[k][0];
            | Group_Y=Returns[k][1];
            | }
        (junction 3309) -> (junction 3311) [order 2]
        (junction 3304) -> (junction 3301) [order 2] : {
            | k=0;
            | j=0;
            | }
        (junction 3356) -> (junction 3358) [order 1] : [(Num_Returns==1) && (Returns[0][2]==0)]%One return, no need to compare
        (junction 3356) -> (junction 3326) [order 2]
        (junction 3358) -> (junction 3360) : {
            | Ini_Tracker_LFSRR_New[Num_Ini_Tracker_LFSRR_New][0]=Returns[0][0];
            | Ini_Tracker_LFSRR_New[Num_Ini_Tracker_LFSRR_New][1]=Returns[0][1];
            | Ini_Tracker_LFSRR_New[Num_Ini_Tracker_LFSRR_New][2]=1;
            | Ini_Tracker_LFSRR_New[Num_Ini_Tracker_LFSRR_New][3]=1;
            | Ini_Tracker_LFSRR_New[Num_Ini_Tracker_LFSRR_New][4]=Returns[0][0];
            | Ini_Tracker_LFSRR_New[Num_Ini_Tracker_LFSRR_New][5]=Returns[0][1];
            | Ini_Tracker_LFSRR_New[Num_Ini_Tracker_LFSRR_New][6]=0;
            | Ini_Tracker_LFSRR_New[Num_Ini_Tracker_LFSRR_New][7]=0;
            | Ini_Tracker_LFSRR_New[Num_Ini_Tracker_LFSRR_New][8]=0;
            | Ini_Tracker_LFSRR_New[Num_Ini_Tracker_LFSRR_New][9]=0;
            | Ini_Tracker_LFSRR_New[Num_Ini_Tracker_LFSRR_New][10]=0;
            | Ini_Tracker_LFSRR_New[Num_Ini_Tracker_LFSRR_New][11]=0;
            | Num_Ini_Tracker_LFSRR_New++;
            | }
        (junction 3330) -> (junction 3311)
        (junction 3328) -> (junction 3330)
        (junction 3314) -> (junction 3334) [order 1] : [Group_Num>0]%There exist more than one near unused returns
        (junction 3334) -> (junction 3342) [order 1] : [n<Group_Num]
        (junction 3344) -> (junction 3334) : {
            | n++;
            | }
        (junction 3352) -> (junction 3303)
        (junction 3314) -> (junction 3349) [order 2]
        (junction 3334) -> (junction 3347) [order 2] : {
            | n=0;
            | Group_X=Group_X/(Group_Num+1);Group_Y=Group_Y/(Group_Num+1);
            | }
        (junction 3342) -> (junction 3344) : {
            | Group_X=Group_X+Group_Data[n][0];
            | Group_Y=Group_Y+Group_Data[n][1];
            | }
        (junction 3347) -> (junction 3349)
        (junction 3349) -> (junction 3336) : {
            | Ini_Tracker_LFSRR_New[Num_Ini_Tracker_LFSRR_New][0]=Group_X;
            | Ini_Tracker_LFSRR_New[Num_Ini_Tracker_LFSRR_New][1]=Group_Y;
            | Ini_Tracker_LFSRR_New[Num_Ini_Tracker_LFSRR_New][2]=1;
            | Ini_Tracker_LFSRR_New[Num_Ini_Tracker_LFSRR_New][3]=1;
            | Ini_Tracker_LFSRR_New[Num_Ini_Tracker_LFSRR_New][4]=Group_X;
            | Ini_Tracker_LFSRR_New[Num_Ini_Tracker_LFSRR_New][5]=Group_Y;
            | Ini_Tracker_LFSRR_New[Num_Ini_Tracker_LFSRR_New][6]=0;
            | Ini_Tracker_LFSRR_New[Num_Ini_Tracker_LFSRR_New][7]=0;
            | Ini_Tracker_LFSRR_New[Num_Ini_Tracker_LFSRR_New][8]=0;
            | Ini_Tracker_LFSRR_New[Num_Ini_Tracker_LFSRR_New][9]=0;
            | Ini_Tracker_LFSRR_New[Num_Ini_Tracker_LFSRR_New][10]=0;
            | Ini_Tracker_LFSRR_New[Num_Ini_Tracker_LFSRR_New][11]=0;
            | Num_Ini_Tracker_LFSRR_New++;
            | }
        (junction 3360) -> (junction 3326)
        (junction 3301) -> (junction 3360)
        (junction 3336) -> (junction 3352)
        (junction 3326) -> (junction 3363)
      (default) -> (junction 1728) : {
          | Ini_Tracker_LFSRR=Ini_Tracker_LFSRR_New;
          | Num_Ini_Tracker_LFSRR=Num_Ini_Tracker_LFSRR_New;
          | Num_Ini_Tracker_LFSRR_New=0;Ini_Tracker_LFSRR_New=0;
          | AssoFlgtm=0;Group_Data=0;Group_Num=0;
          | }
      (junction 1728) -> (junction 1730) [order 1] : [k<30]
      (junction 1730) -> (junction 1736) [order 1] : [Ini_Tracker_LFSRR[k][2]>0]
      (junction 1740) -> (junction 1728) : {
          | k++;
          | }
      (junction 1728) -> (junction 1744) [order 2] : {
          | k=0;
          | }
      (junction 1730) -> (junction 1740) [order 2]
      (junction 1736) -> (junction 1738) : {
          | LFSRR_Ini_Update();
          | }
      (junction 1738) -> (junction 1740)
      (junction 1744) -> (junction 1892) : {
          | LFFirstTrackGen();
          | }
    state RFSRR_Ini [function]
      state RFSRR_Ini_Update [function]
        note: %Recently used in 4/5 logical modle in the initial of radar tracker
        state Ini_FifthTime_RF [function]
          (default) -> (junction 2177) : {
              | RelDeg=0;Min_Distance_IniTrack=9;RelativeDist=0;
              | x_5_predict=3*Ini_Tracker_RFSRR[k][10]-3*Ini_Tracker_RFSRR[k][8]+Ini_Tracker_RFSRR[k][6];%Use three point to predict next point based constant acc
              | y_5_predict=3*Ini_Tracker_RFSRR[k][11]-3*Ini_Tracker_RFSRR[k][9]+Ini_Tracker_RFSRR[k][7];%Use three point to predict next point based constant acc
              | Updatereturn=0;Ini_Tracker_UpdateFlg=0;
              | }
          (junction 2177) -> (junction 2905) [order 1] : [(j<Num_Returns)]
          (junction 2905) -> (junction 2178) [order 1] : [Returns[j][2]==0]
          (junction 2907) -> (junction 2177) : {
              | j++;
              | }
          (junction 2178) -> (junction 2179) : {
              | RelativeDist=(x_5_predict-Returns[j][0])*(x_5_predict-Returns[j][0])+(y_5_predict-Returns[j][1])*(y_5_predict-Returns[j][1]);
              | RelDeg=cos_cal(Ini_Tracker_RFSRR[k][8],Ini_Tracker_RFSRR[k][9],...
              | Ini_Tracker_RFSRR[k][10],Ini_Tracker_RFSRR[k][11],Returns[j][0],Returns[j][1]);
              | }
          (junction 2177) -> (junction 2185) [order 2] : {
              | j=0;
              | }
          (junction 2905) -> (junction 2907) [order 2]
          (junction 2179) -> (junction 3047) [order 1] : [(RelativeDist<4)]
          (junction 3047) -> (junction 3050) [order 1] : [(RelativeDist<0.1)]
          (junction 2179) -> (junction 2182) [order 2]
          (junction 3047) -> (junction 3051) [order 2]
          (junction 3050) -> (junction 3033)
          (junction 3051) -> (junction 3033) [order 1] : [(((RelDeg>120) || (RelDeg<60)))]
          (junction 3033) -> (junction 3037) [order 1] : [RelativeDist<Min_Distance_IniTrack]
          (junction 3051) -> (junction 3045) [order 2]
          (junction 3033) -> (junction 3041) [order 2]
          (junction 3037) -> (junction 3039) : {
              | Updatereturn=j;
              | Ini_Tracker_UpdateFlg=1;
              | Min_Distance_IniTrack=RelativeDist;
              | }
          (junction 2182) -> (junction 2907)
          (junction 3045) -> (junction 2182)
          (junction 3041) -> (junction 3045)
          (junction 3039) -> (junction 3041)
          (junction 2185) -> (junction 2186) [order 1] : [Ini_Tracker_UpdateFlg==1]%Means that the tracker k found measurement
          (junction 2185) -> (junction 2187) [order 2] : {
              | %cound not found, and enter 5 searches means that could not found once before, so delete
              | }
          (junction 2186) -> (junction 2188) : {
              | Returns[Updatereturn][2]=1;
              | %Which means that the return is used
              | TrackIni(Returns[Updatereturn][0],Returns[Updatereturn][1]);
              | }
          (junction 2188) -> (junction 2187)
          (junction 2187) -> (junction 2189) : {
              | Updatereturn=0;Ini_Tracker_UpdateFlg=0;
              | }
        state Ini_ForthTime_RF [function]
          (default) -> (junction 2208) : {
              | RelDeg=0;Min_Distance_IniTrack=9;RelativeDist=0;
              | x_4_predict=3*Ini_Tracker_RFSRR[k][8]-3*Ini_Tracker_RFSRR[k][6]+Ini_Tracker_RFSRR[k][4];%Use three point to predict next point based constant acc
              | y_4_predict=3*Ini_Tracker_RFSRR[k][9]-3*Ini_Tracker_RFSRR[k][7]+Ini_Tracker_RFSRR[k][5];%Use three point to predict next point based constant acc
              | Updatereturn=0;Ini_Tracker_UpdateFlg=0;
              | }
          (junction 2208) -> (junction 2900) [order 1] : [(j<Num_Returns)]
          (junction 2900) -> (junction 2209) [order 1] : [(Returns[j][2]==0)]
          (junction 2902) -> (junction 2208) : {
              | j++;
              | }
          (junction 2209) -> (junction 2210) : {
              | RelativeDist=(x_4_predict-Returns[j][0])*(x_4_predict-Returns[j][0])+(y_4_predict-Returns[j][1])*(y_4_predict-Returns[j][1]);
              | RelDeg=cos_cal(Ini_Tracker_RFSRR[k][6],Ini_Tracker_RFSRR[k][7],...
              | Ini_Tracker_RFSRR[k][8],Ini_Tracker_RFSRR[k][9],Returns[j][0],Returns[j][1]);
              | }
          (junction 2208) -> (junction 2216) [order 2] : {
              | j=0;
              | }
          (junction 2900) -> (junction 2902) [order 2]
          (junction 2210) -> (junction 3027) [order 1] : [(RelativeDist<4)]
          (junction 3027) -> (junction 3030) [order 1] : [(RelativeDist<0.1)]
          (junction 2210) -> (junction 2213) [order 2]
          (junction 3027) -> (junction 3031) [order 2]
          (junction 3030) -> (junction 3013)
          (junction 3031) -> (junction 3013) [order 1] : [(((RelDeg>120) || (RelDeg<60)))]
          (junction 3013) -> (junction 3017) [order 1] : [RelativeDist<Min_Distance_IniTrack]
          (junction 3031) -> (junction 3025) [order 2]
          (junction 3013) -> (junction 3021) [order 2]
          (junction 3017) -> (junction 3019) : {
              | Updatereturn=j;
              | Ini_Tracker_UpdateFlg=1;
              | Min_Distance_IniTrack=RelativeDist;
              | }
          (junction 2213) -> (junction 2902)
          (junction 3025) -> (junction 2213)
          (junction 3021) -> (junction 3025)
          (junction 3019) -> (junction 3021)
          (junction 2216) -> (junction 2217) [order 1] : [Ini_Tracker_UpdateFlg==1]%Means that the tracker k found measurement
          (junction 2217) -> (junction 2218) [order 1] : [Ini_Tracker_RFSRR[k][3]==3]%Has found measurement 4 times and begin ini
          (junction 2216) -> (junction 2220) [order 2]
          (junction 2217) -> (junction 2223) [order 2] : {
              | Returns[Updatereturn][2]=1;%Which means that the return is used
              | Ini_Tracker_RFSRR_New[Num_Ini_Tracker_RFSRR_New][0]=Returns[Updatereturn][0];
              | Ini_Tracker_RFSRR_New[Num_Ini_Tracker_RFSRR_New][1]=Returns[Updatereturn][1];
              | Ini_Tracker_RFSRR_New[Num_Ini_Tracker_RFSRR_New][2]=4;%Tracker counter
              | Ini_Tracker_RFSRR_New[Num_Ini_Tracker_RFSRR_New][3]=3;%Association counter
              | Ini_Tracker_RFSRR_New[Num_Ini_Tracker_RFSRR_New][4]=Ini_Tracker_RFSRR[k][4];
              | Ini_Tracker_RFSRR_New[Num_Ini_Tracker_RFSRR_New][5]=Ini_Tracker_RFSRR[k][5];
              | Ini_Tracker_RFSRR_New[Num_Ini_Tracker_RFSRR_New][6]=Ini_Tracker_RFSRR[k][6];
              | Ini_Tracker_RFSRR_New[Num_Ini_Tracker_RFSRR_New][7]=Ini_Tracker_RFSRR[k][7];
              | Ini_Tracker_RFSRR_New[Num_Ini_Tracker_RFSRR_New][8]=Ini_Tracker_RFSRR[k][8];
              | Ini_Tracker_RFSRR_New[Num_Ini_Tracker_RFSRR_New][9]=Ini_Tracker_RFSRR[k][9];
              | Ini_Tracker_RFSRR_New[Num_Ini_Tracker_RFSRR_New][10]=Returns[Updatereturn][0];
              | Ini_Tracker_RFSRR_New[Num_Ini_Tracker_RFSRR_New][11]=Returns[Updatereturn][1];
              | Num_Ini_Tracker_RFSRR_New++;
              | }
          (junction 2218) -> (junction 2224) : {
              | Returns[Updatereturn][2]=1;
              | %Which means that the return is used
              | TrackIni(Returns[Updatereturn][0],Returns[Updatereturn][1]);
              | }
          (junction 2220) -> (junction 2219) [order 1] : [Ini_Tracker_RFSRR[k][3]==3]
              | %Has found measurement 3 times before
          (junction 2219) -> (junction 2222) : {
              | Ini_Tracker_RFSRR_New[Num_Ini_Tracker_RFSRR_New][0]=x_4_predict;
              | Ini_Tracker_RFSRR_New[Num_Ini_Tracker_RFSRR_New][1]=y_4_predict;
              | Ini_Tracker_RFSRR_New[Num_Ini_Tracker_RFSRR_New][2]=4;%Tracker counter
              | Ini_Tracker_RFSRR_New[Num_Ini_Tracker_RFSRR_New][3]=3;%Association counter
              | Ini_Tracker_RFSRR_New[Num_Ini_Tracker_RFSRR_New][4]=Ini_Tracker_RFSRR[k][4];
              | Ini_Tracker_RFSRR_New[Num_Ini_Tracker_RFSRR_New][5]=Ini_Tracker_RFSRR[k][5];
              | Ini_Tracker_RFSRR_New[Num_Ini_Tracker_RFSRR_New][6]=Ini_Tracker_RFSRR[k][6];
              | Ini_Tracker_RFSRR_New[Num_Ini_Tracker_RFSRR_New][7]=Ini_Tracker_RFSRR[k][7];
              | Ini_Tracker_RFSRR_New[Num_Ini_Tracker_RFSRR_New][8]=Ini_Tracker_RFSRR[k][8];
              | Ini_Tracker_RFSRR_New[Num_Ini_Tracker_RFSRR_New][9]=Ini_Tracker_RFSRR[k][9];
              | Ini_Tracker_RFSRR_New[Num_Ini_Tracker_RFSRR_New][10]=x_4_predict;
              | Ini_Tracker_RFSRR_New[Num_Ini_Tracker_RFSRR_New][11]=y_4_predict;
              | Num_Ini_Tracker_RFSRR_New++;
              | }
          (junction 2220) -> (junction 2221) [order 2] : {
              | %Cound not found measurement twice,
              | % So not transfer tracker k to new list
              | }
          (junction 2222) -> (junction 2221)
          (junction 2223) -> (junction 2222)
          (junction 2224) -> (junction 2223)
          (junction 2221) -> (junction 2225) : {
              | Updatereturn=0;Ini_Tracker_UpdateFlg=0;
              | }
        state Ini_ThridTime_RF [function]
          (default) -> (junction 2251) : {
              | RelDeg=0;Min_Distance_IniTrack=9;RelativeDist=0;
              | x_3_predict=2*Ini_Tracker_RFSRR[k][6]-Ini_Tracker_RFSRR[k][4];%Use two point to predict next point based constant velocity
              | y_3_predict=2*Ini_Tracker_RFSRR[k][7]-Ini_Tracker_RFSRR[k][5];%Use two point to predict next point based constant velocity
              | Updatereturn=0;Ini_Tracker_UpdateFlg=0;
              | }
          (junction 2251) -> (junction 2895) [order 1] : [(j<Num_Returns)]
          (junction 2895) -> (junction 2252) [order 1] : [(Returns[j][2]==0)]
          (junction 2897) -> (junction 2251) : {
              | j++;
              | }
          (junction 2252) -> (junction 2253) : {
              | RelativeDist=(x_3_predict-Returns[j][0])*(x_3_predict-Returns[j][0])+(y_3_predict-Returns[j][1])*(y_3_predict-Returns[j][1]);
              | RelDeg=cos_cal(Ini_Tracker_RFSRR[k][4],Ini_Tracker_RFSRR[k][5],...
              | Ini_Tracker_RFSRR[k][6],Ini_Tracker_RFSRR[k][7],Returns[j][0],Returns[j][1]);
              | }
          (junction 2251) -> (junction 2259) [order 2] : {
              | j=0;
              | }
          (junction 2895) -> (junction 2897) [order 2]
          (junction 2253) -> (junction 3007) [order 1] : [(RelativeDist<4)]
          (junction 3007) -> (junction 3010) [order 1] : [(RelativeDist<0.1)]
          (junction 2253) -> (junction 2256) [order 2]
          (junction 3007) -> (junction 3011) [order 2]
          (junction 3010) -> (junction 2993)
          (junction 3011) -> (junction 2993) [order 1] : [(((RelDeg>120) || (RelDeg<60)))]
          (junction 2993) -> (junction 2997) [order 1] : [RelativeDist<Min_Distance_IniTrack]
          (junction 3011) -> (junction 3005) [order 2]
          (junction 2993) -> (junction 3001) [order 2]
          (junction 2997) -> (junction 2999) : {
              | Updatereturn=j;
              | Ini_Tracker_UpdateFlg=1;
              | Min_Distance_IniTrack=RelativeDist;
              | }
          (junction 2256) -> (junction 2897)
          (junction 3005) -> (junction 2256)
          (junction 3001) -> (junction 3005)
          (junction 2999) -> (junction 3001)
          (junction 2259) -> (junction 2260) [order 1] : [Ini_Tracker_UpdateFlg==1]%Means that the tracker k found measurement
          (junction 2259) -> (junction 2261) [order 2] : {
              | Ini_Tracker_RFSRR_New[Num_Ini_Tracker_RFSRR_New][0]=x_3_predict;
              | Ini_Tracker_RFSRR_New[Num_Ini_Tracker_RFSRR_New][1]=y_3_predict;
              | Ini_Tracker_RFSRR_New[Num_Ini_Tracker_RFSRR_New][2]=3;%Tracker counter
              | Ini_Tracker_RFSRR_New[Num_Ini_Tracker_RFSRR_New][3]=2;%Association counter
              | Ini_Tracker_RFSRR_New[Num_Ini_Tracker_RFSRR_New][4]=Ini_Tracker_RFSRR[k][4];
              | Ini_Tracker_RFSRR_New[Num_Ini_Tracker_RFSRR_New][5]=Ini_Tracker_RFSRR[k][5];
              | Ini_Tracker_RFSRR_New[Num_Ini_Tracker_RFSRR_New][6]=Ini_Tracker_RFSRR[k][6];
              | Ini_Tracker_RFSRR_New[Num_Ini_Tracker_RFSRR_New][7]=Ini_Tracker_RFSRR[k][7];
              | Ini_Tracker_RFSRR_New[Num_Ini_Tracker_RFSRR_New][8]=x_3_predict;
              | Ini_Tracker_RFSRR_New[Num_Ini_Tracker_RFSRR_New][9]=y_3_predict;
              | Num_Ini_Tracker_RFSRR_New++;
              | }
          (junction 2260) -> (junction 2262) : {
              | Returns[Updatereturn][2]=1;%Which means that the return is used
              | Ini_Tracker_RFSRR_New[Num_Ini_Tracker_RFSRR_New][0]=Returns[Updatereturn][0];
              | Ini_Tracker_RFSRR_New[Num_Ini_Tracker_RFSRR_New][1]=Returns[Updatereturn][1];
              | Ini_Tracker_RFSRR_New[Num_Ini_Tracker_RFSRR_New][2]=3;%Tracker counter
              | Ini_Tracker_RFSRR_New[Num_Ini_Tracker_RFSRR_New][3]=3;%Association counter
              | Ini_Tracker_RFSRR_New[Num_Ini_Tracker_RFSRR_New][4]=Ini_Tracker_RFSRR[k][4];
              | Ini_Tracker_RFSRR_New[Num_Ini_Tracker_RFSRR_New][5]=Ini_Tracker_RFSRR[k][5];
              | Ini_Tracker_RFSRR_New[Num_Ini_Tracker_RFSRR_New][6]=Ini_Tracker_RFSRR[k][6];
              | Ini_Tracker_RFSRR_New[Num_Ini_Tracker_RFSRR_New][7]=Ini_Tracker_RFSRR[k][7];
              | Ini_Tracker_RFSRR_New[Num_Ini_Tracker_RFSRR_New][8]=Returns[Updatereturn][0];
              | Ini_Tracker_RFSRR_New[Num_Ini_Tracker_RFSRR_New][9]=Returns[Updatereturn][1];
              | Num_Ini_Tracker_RFSRR_New++;
              | }
          (junction 2262) -> (junction 2261)
          (junction 2261) -> (junction 2263) : {
              | Updatereturn=0;Ini_Tracker_UpdateFlg=0;
              | }
        state Ini_SecondTime_RF [function]
          (default) -> (junction 2282) : {
              | AssoFlgtm=0;
              | }
          (junction 2282) -> (junction 2283) [order 1] : [j<Num_Returns]
          (junction 2284) -> (junction 2282) : {
              | j++;
              | }
          (junction 2283) -> (junction 2284) : {
              | AssoFlgtm[j]=VelocityMethod(Ini_Tracker_RFSRR[k][4],Ini_Tracker_RFSRR[k][5],...
              | Returns[j][0],Returns[j][1],10,0,5,0,1.5,1.5,5,0.04);%Velocity Association method
              | }
          (junction 2282) -> (junction 2285) [order 2] : {
              | j=0;
              | }
          (junction 2285) -> (junction 2286) [order 1] : [j<Num_Returns]
          (junction 2286) -> (junction 2287) [order 1] : [AssoFlgtm[j]==1]
          (junction 2288) -> (junction 2285) : {
              | j++;
              | }
          (junction 2285) -> (junction 2290) [order 2] : {
              | j=0;
              | AssoFlgtm=0;
              | }
          (junction 2286) -> (junction 2288) [order 2]
          (junction 2287) -> (junction 2289) : {
              | Returns[j][2]=1;%Which means that the return is used
              | Ini_Tracker_RFSRR_New[Num_Ini_Tracker_RFSRR_New][0]=Returns[j][0];
              | Ini_Tracker_RFSRR_New[Num_Ini_Tracker_RFSRR_New][1]=Returns[j][1];
              | Ini_Tracker_RFSRR_New[Num_Ini_Tracker_RFSRR_New][2]=2;
              | Ini_Tracker_RFSRR_New[Num_Ini_Tracker_RFSRR_New][3]=2;
              | Ini_Tracker_RFSRR_New[Num_Ini_Tracker_RFSRR_New][4]=Ini_Tracker_RFSRR[k][4];
              | Ini_Tracker_RFSRR_New[Num_Ini_Tracker_RFSRR_New][5]=Ini_Tracker_RFSRR[k][5];
              | Ini_Tracker_RFSRR_New[Num_Ini_Tracker_RFSRR_New][6]=Returns[j][0];
              | Ini_Tracker_RFSRR_New[Num_Ini_Tracker_RFSRR_New][7]=Returns[j][1];
              | Num_Ini_Tracker_RFSRR_New++;
              | }
          (junction 2289) -> (junction 2288)
        (default) -> (junction 2137)
        (junction 2137) -> (junction 2138) [order 1] : [Ini_Tracker_RFSRR[k][2]==4]%This Tracker has updated forth and find fifth measurement
        (junction 2137) -> (junction 2139) [order 2]
        (junction 2138) -> (junction 2140) : {
            | Ini_FifthTime_RF();
            | }
        (junction 2140) -> (junction 2139)
        (junction 2139) -> (junction 2141)
        (junction 2141) -> (junction 2142) [order 1] : [Ini_Tracker_RFSRR[k][2]==3]%This Tracker has updated thrid and find forth measurement
        (junction 2141) -> (junction 2143) [order 2]
        (junction 2142) -> (junction 2144) : {
            | Ini_ForthTime_RF();
            | }
        (junction 2144) -> (junction 2143)
        (junction 2143) -> (junction 2145)
        (junction 2145) -> (junction 2146) [order 1] : [Ini_Tracker_RFSRR[k][2]==2]%This Tracker has updated once and find thrid measurement
        (junction 2145) -> (junction 2147) [order 2]
        (junction 2146) -> (junction 2148) : {
            | Ini_ThridTime_RF();
            | }
        (junction 2148) -> (junction 2147)
        (junction 2147) -> (junction 2149)
        (junction 2149) -> (junction 2150) [order 1] : [Ini_Tracker_RFSRR[k][2]==1]%This Tracker is first initial and use velocity to find next measurements
        (junction 2149) -> (junction 2151) [order 2]
        (junction 2150) -> (junction 2152) : {
            | Ini_SecondTime_RF();
            | }
        (junction 2152) -> (junction 2151)
        (junction 2151) -> (junction 2153)
      state RFFirstTrackGen [function]
        (default) -> (junction 3376)
        (junction 3376) -> (junction 3377) [order 1] : [Num_Returns>1]%Two return, begine compare
        (junction 3376) -> (junction 3384) [order 2]
        (junction 3377) -> (junction 3383) : {
            | j=1;
            | }
        (junction 3378) -> (junction 3379) [order 1] : [(Returns[k][0]-Returns[j][0])*(Returns[k][0]-Returns[j][0])+...
            | (Returns[k][1]-Returns[j][1])*(Returns[k][1]-Returns[j][1])<=9]
        (junction 3382) -> (junction 3378) [order 1] : [Returns[j][2]==0]
        (junction 3380) -> (junction 3381) [order 1] : [Returns[k][2]==0]
        (junction 3381) -> (junction 3382) [order 1] : [j<Num_Returns]
        (junction 3383) -> (junction 3380) [order 1] : [k<Num_Returns-1]
        (junction 3386) -> (junction 3381) : {
            | j++;
            | }
        (junction 3378) -> (junction 3387) [order 2]
        (junction 3379) -> (junction 3388) : {
            | Group_Data[Group_Num][0]=Returns[j][0];
            | Group_Data[Group_Num][1]=Returns[j][1];
            | Returns[j][2]=1;
            | Group_Num=Group_Num+1;
            | }
        (junction 3389) -> (junction 3383) : {
            | k++;
            | j=k+1;
            | Group_Num=0;
            | Group_Data=0;
            | Group_X=0;
            | Group_Y=0;
            | }
        (junction 3380) -> (junction 3389) [order 2]
        (junction 3381) -> (junction 3390) [order 2] : {
            | Group_X=Returns[k][0];
            | Group_Y=Returns[k][1];
            | }
        (junction 3382) -> (junction 3386) [order 2]
        (junction 3383) -> (junction 3398) [order 2] : {
            | k=0;
            | j=0;
            | }
        (junction 3384) -> (junction 3385) [order 1] : [(Num_Returns==1) && (Returns[0][2]==0)]%One return, no need to compare
        (junction 3384) -> (junction 3396) [order 2]
        (junction 3385) -> (junction 3397) : {
            | Ini_Tracker_RFSRR_New[Num_Ini_Tracker_RFSRR_New][0]=Returns[0][0];
            | Ini_Tracker_RFSRR_New[Num_Ini_Tracker_RFSRR_New][1]=Returns[0][1];
            | Ini_Tracker_RFSRR_New[Num_Ini_Tracker_RFSRR_New][2]=1;
            | Ini_Tracker_RFSRR_New[Num_Ini_Tracker_RFSRR_New][3]=1;
            | Ini_Tracker_RFSRR_New[Num_Ini_Tracker_RFSRR_New][4]=Returns[0][0];
            | Ini_Tracker_RFSRR_New[Num_Ini_Tracker_RFSRR_New][5]=Returns[0][1];
            | Ini_Tracker_RFSRR_New[Num_Ini_Tracker_RFSRR_New][6]=0;
            | Ini_Tracker_RFSRR_New[Num_Ini_Tracker_RFSRR_New][7]=0;
            | Ini_Tracker_RFSRR_New[Num_Ini_Tracker_RFSRR_New][8]=0;
            | Ini_Tracker_RFSRR_New[Num_Ini_Tracker_RFSRR_New][9]=0;
            | Ini_Tracker_RFSRR_New[Num_Ini_Tracker_RFSRR_New][10]=0;
            | Ini_Tracker_RFSRR_New[Num_Ini_Tracker_RFSRR_New][11]=0;
            | Num_Ini_Tracker_RFSRR_New++;
            | }
        (junction 3387) -> (junction 3386)
        (junction 3388) -> (junction 3387)
        (junction 3390) -> (junction 3391) [order 1] : [Group_Num>0]%There exist more than one near unused returns
        (junction 3391) -> (junction 3392) [order 1] : [n<Group_Num]
        (junction 3393) -> (junction 3391) : {
            | n++;
            | }
        (junction 3399) -> (junction 3389)
        (junction 3390) -> (junction 3394) [order 2]
        (junction 3391) -> (junction 3395) [order 2] : {
            | n=0;
            | Group_X=Group_X/(Group_Num+1);Group_Y=Group_Y/(Group_Num+1);
            | }
        (junction 3392) -> (junction 3393) : {
            | Group_X=Group_X+Group_Data[n][0];
            | Group_Y=Group_Y+Group_Data[n][1];
            | }
        (junction 3395) -> (junction 3394)
        (junction 3394) -> (junction 3400) : {
            | Ini_Tracker_RFSRR_New[Num_Ini_Tracker_RFSRR_New][0]=Group_X;
            | Ini_Tracker_RFSRR_New[Num_Ini_Tracker_RFSRR_New][1]=Group_Y;
            | Ini_Tracker_RFSRR_New[Num_Ini_Tracker_RFSRR_New][2]=1;
            | Ini_Tracker_RFSRR_New[Num_Ini_Tracker_RFSRR_New][3]=1;
            | Ini_Tracker_RFSRR_New[Num_Ini_Tracker_RFSRR_New][4]=Group_X;
            | Ini_Tracker_RFSRR_New[Num_Ini_Tracker_RFSRR_New][5]=Group_Y;
            | Ini_Tracker_RFSRR_New[Num_Ini_Tracker_RFSRR_New][6]=0;
            | Ini_Tracker_RFSRR_New[Num_Ini_Tracker_RFSRR_New][7]=0;
            | Ini_Tracker_RFSRR_New[Num_Ini_Tracker_RFSRR_New][8]=0;
            | Ini_Tracker_RFSRR_New[Num_Ini_Tracker_RFSRR_New][9]=0;
            | Ini_Tracker_RFSRR_New[Num_Ini_Tracker_RFSRR_New][10]=0;
            | Ini_Tracker_RFSRR_New[Num_Ini_Tracker_RFSRR_New][11]=0;
            | Num_Ini_Tracker_RFSRR_New++;
            | }
        (junction 3397) -> (junction 3396)
        (junction 3398) -> (junction 3397)
        (junction 3400) -> (junction 3399)
        (junction 3396) -> (junction 3401)
      (default) -> (junction 2308) : {
          | Ini_Tracker_RFSRR=Ini_Tracker_RFSRR_New;
          | Num_Ini_Tracker_RFSRR=Num_Ini_Tracker_RFSRR_New;
          | Num_Ini_Tracker_RFSRR_New=0;Ini_Tracker_RFSRR_New=0;
          | AssoFlgtm=0;Group_Data=0;Group_Num=0;
          | }
      (junction 2308) -> (junction 2307) [order 1] : [k<30]
      (junction 2307) -> (junction 2312) [order 1] : [Ini_Tracker_RFSRR[k][2]>0]
      (junction 2311) -> (junction 2308) : {
          | k++;
          | }
      (junction 2308) -> (junction 2314) [order 2] : {
          | k=0;
          | }
      (junction 2307) -> (junction 2311) [order 2]
      (junction 2312) -> (junction 2315) : {
          | RFSRR_Ini_Update();
          | }
      (junction 2315) -> (junction 2311)
      (junction 2314) -> (junction 2318) : {
          | RFFirstTrackGen();
          | }
    state LRSRR_Ini [function]
      state LRSRR_Ini_Update [function]
        note: %Recently used in 4/5 logical modle in the initial of radar tracker
        state Ini_FifthTime_LR [function]
          (default) -> (junction 2387) : {
              | RelDeg=0;Min_Distance_IniTrack=9;RelativeDist=0;
              | x_5_predict=3*Ini_Tracker_LRSRR[k][10]-3*Ini_Tracker_LRSRR[k][8]+Ini_Tracker_LRSRR[k][6];%Use three point to predict next point based constant acc
              | y_5_predict=3*Ini_Tracker_LRSRR[k][11]-3*Ini_Tracker_LRSRR[k][9]+Ini_Tracker_LRSRR[k][7];%Use three point to predict next point based constant acc
              | Updatereturn=0;Ini_Tracker_UpdateFlg=0;
              | }
          (junction 2920) -> (junction 2388) [order 1] : [(Returns[j][2]==0)]
          (junction 2387) -> (junction 2920) [order 1] : [(j<Num_Returns)]
          (junction 2922) -> (junction 2387) : {
              | j++;
              | }
          (junction 2388) -> (junction 2389) : {
              | RelativeDist=(x_5_predict-Returns[j][0])*(x_5_predict-Returns[j][0])+(y_5_predict-Returns[j][1])*(y_5_predict-Returns[j][1]);
              | RelDeg=cos_cal(Ini_Tracker_LRSRR[k][8],Ini_Tracker_LRSRR[k][9],...
              | Ini_Tracker_LRSRR[k][10],Ini_Tracker_LRSRR[k][11],Returns[j][0],Returns[j][1]);
              | }
          (junction 2387) -> (junction 2395) [order 2] : {
              | j=0;
              | }
          (junction 2920) -> (junction 2922) [order 2]
          (junction 2389) -> (junction 3107) [order 1] : [(RelativeDist<4)]
          (junction 3107) -> (junction 3110) [order 1] : [(RelativeDist<0.1)]
          (junction 2389) -> (junction 2392) [order 2]
          (junction 3107) -> (junction 3111) [order 2]
          (junction 3110) -> (junction 3093)
          (junction 3111) -> (junction 3093) [order 1] : [(((RelDeg>120) || (RelDeg<60)))]
          (junction 3093) -> (junction 3097) [order 1] : [RelativeDist<Min_Distance_IniTrack]
          (junction 3111) -> (junction 3105) [order 2]
          (junction 3093) -> (junction 3101) [order 2]
          (junction 3097) -> (junction 3099) : {
              | Updatereturn=j;
              | Ini_Tracker_UpdateFlg=1;
              | Min_Distance_IniTrack=RelativeDist;
              | }
          (junction 2392) -> (junction 2922)
          (junction 3105) -> (junction 2392)
          (junction 3101) -> (junction 3105)
          (junction 3099) -> (junction 3101)
          (junction 2395) -> (junction 2396) [order 1] : [Ini_Tracker_UpdateFlg==1]%Means that the tracker k found measurement
          (junction 2395) -> (junction 2397) [order 2] : {
              | %cound not found, and enter 5 searches means that could not found once before, so delete
              | }
          (junction 2396) -> (junction 2398) : {
              | Returns[Updatereturn][2]=1;
              | %Which means that the return is used
              | TrackIni(Returns[Updatereturn][0],Returns[Updatereturn][1]);
              | }
          (junction 2398) -> (junction 2397)
          (junction 2397) -> (junction 2399) : {
              | Updatereturn=0;Ini_Tracker_UpdateFlg=0;
              | }
        state Ini_ForthTime_LR [function]
          (default) -> (junction 2418) : {
              | RelDeg=0;Min_Distance_IniTrack=9;RelativeDist=0;
              | x_4_predict=3*Ini_Tracker_LRSRR[k][8]-3*Ini_Tracker_LRSRR[k][6]+Ini_Tracker_LRSRR[k][4];%Use three point to predict next point based constant acc
              | y_4_predict=3*Ini_Tracker_LRSRR[k][9]-3*Ini_Tracker_LRSRR[k][7]+Ini_Tracker_LRSRR[k][5];%Use three point to predict next point based constant acc
              | Updatereturn=0;Ini_Tracker_UpdateFlg=0;
              | }
          (junction 2418) -> (junction 2915) [order 1] : [(j<Num_Returns)]
          (junction 2915) -> (junction 2419) [order 1] : [(Returns[j][2]==0)]
          (junction 2917) -> (junction 2418) : {
              | j++;
              | }
          (junction 2418) -> (junction 2426) [order 2] : {
              | j=0;
              | }
          (junction 2915) -> (junction 2917) [order 2]
          (junction 2419) -> (junction 2420) : {
              | RelativeDist=(x_4_predict-Returns[j][0])*(x_4_predict-Returns[j][0])+(y_4_predict-Returns[j][1])*(y_4_predict-Returns[j][1]);
              | RelDeg=cos_cal(Ini_Tracker_LRSRR[k][6],Ini_Tracker_LRSRR[k][7],...
              | Ini_Tracker_LRSRR[k][8],Ini_Tracker_LRSRR[k][9],Returns[j][0],Returns[j][1]);
              | }
          (junction 2420) -> (junction 3087) [order 1] : [(RelativeDist<4)]
          (junction 3087) -> (junction 3090) [order 1] : [(RelativeDist<0.1)]
          (junction 2420) -> (junction 2423) [order 2]
          (junction 3087) -> (junction 3091) [order 2]
          (junction 3090) -> (junction 3073)
          (junction 3091) -> (junction 3073) [order 1] : [(((RelDeg>120) || (RelDeg<60)))]
          (junction 3073) -> (junction 3077) [order 1] : [RelativeDist<Min_Distance_IniTrack]
          (junction 3091) -> (junction 3085) [order 2]
          (junction 3073) -> (junction 3081) [order 2]
          (junction 3077) -> (junction 3079) : {
              | Updatereturn=j;
              | Ini_Tracker_UpdateFlg=1;
              | Min_Distance_IniTrack=RelativeDist;
              | }
          (junction 2423) -> (junction 2917)
          (junction 3085) -> (junction 2423)
          (junction 3081) -> (junction 3085)
          (junction 3079) -> (junction 3081)
          (junction 2426) -> (junction 2427) [order 1] : [Ini_Tracker_UpdateFlg==1]%Means that the tracker k found measurement
          (junction 2427) -> (junction 2428) [order 1] : [Ini_Tracker_LRSRR[k][3]==3]%Has found measurement 4 times and begin ini
          (junction 2426) -> (junction 2430) [order 2]
          (junction 2427) -> (junction 2433) [order 2] : {
              | Returns[Updatereturn][2]=1;%Which means that the return is used
              | Ini_Tracker_LRSRR_New[Num_Ini_Tracker_LRSRR_New][0]=Returns[Updatereturn][0];
              | Ini_Tracker_LRSRR_New[Num_Ini_Tracker_LRSRR_New][1]=Returns[Updatereturn][1];
              | Ini_Tracker_LRSRR_New[Num_Ini_Tracker_LRSRR_New][2]=4;%Tracker counter
              | Ini_Tracker_LRSRR_New[Num_Ini_Tracker_LRSRR_New][3]=3;%Association counter
              | Ini_Tracker_LRSRR_New[Num_Ini_Tracker_LRSRR_New][4]=Ini_Tracker_LRSRR[k][4];
              | Ini_Tracker_LRSRR_New[Num_Ini_Tracker_LRSRR_New][5]=Ini_Tracker_LRSRR[k][5];
              | Ini_Tracker_LRSRR_New[Num_Ini_Tracker_LRSRR_New][6]=Ini_Tracker_LRSRR[k][6];
              | Ini_Tracker_LRSRR_New[Num_Ini_Tracker_LRSRR_New][7]=Ini_Tracker_LRSRR[k][7];
              | Ini_Tracker_LRSRR_New[Num_Ini_Tracker_LRSRR_New][8]=Ini_Tracker_LRSRR[k][8];
              | Ini_Tracker_LRSRR_New[Num_Ini_Tracker_LRSRR_New][9]=Ini_Tracker_LRSRR[k][9];
              | Ini_Tracker_LRSRR_New[Num_Ini_Tracker_LRSRR_New][10]=Returns[Updatereturn][0];
              | Ini_Tracker_LRSRR_New[Num_Ini_Tracker_LRSRR_New][11]=Returns[Updatereturn][1];
              | Num_Ini_Tracker_LRSRR_New++;
              | }
          (junction 2428) -> (junction 2434) : {
              | Returns[Updatereturn][2]=1;
              | %Which means that the return is used
              | TrackIni(Returns[Updatereturn][0],Returns[Updatereturn][1]);
              | }
          (junction 2430) -> (junction 2429) [order 1] : [Ini_Tracker_LRSRR[k][3]==3]
              | %Has found measurement 3 times before
          (junction 2429) -> (junction 2432) : {
              | Ini_Tracker_LRSRR_New[Num_Ini_Tracker_LRSRR_New][0]=x_4_predict;
              | Ini_Tracker_LRSRR_New[Num_Ini_Tracker_LRSRR_New][1]=y_4_predict;
              | Ini_Tracker_LRSRR_New[Num_Ini_Tracker_LRSRR_New][2]=4;%Tracker counter
              | Ini_Tracker_LRSRR_New[Num_Ini_Tracker_LRSRR_New][3]=3;%Association counter
              | Ini_Tracker_LRSRR_New[Num_Ini_Tracker_LRSRR_New][4]=Ini_Tracker_LRSRR[k][4];
              | Ini_Tracker_LRSRR_New[Num_Ini_Tracker_LRSRR_New][5]=Ini_Tracker_LRSRR[k][5];
              | Ini_Tracker_LRSRR_New[Num_Ini_Tracker_LRSRR_New][6]=Ini_Tracker_LRSRR[k][6];
              | Ini_Tracker_LRSRR_New[Num_Ini_Tracker_LRSRR_New][7]=Ini_Tracker_LRSRR[k][7];
              | Ini_Tracker_LRSRR_New[Num_Ini_Tracker_LRSRR_New][8]=Ini_Tracker_LRSRR[k][8];
              | Ini_Tracker_LRSRR_New[Num_Ini_Tracker_LRSRR_New][9]=Ini_Tracker_LRSRR[k][9];
              | Ini_Tracker_LRSRR_New[Num_Ini_Tracker_LRSRR_New][10]=x_4_predict;
              | Ini_Tracker_LRSRR_New[Num_Ini_Tracker_LRSRR_New][11]=y_4_predict;
              | Num_Ini_Tracker_LRSRR_New++;
              | }
          (junction 2430) -> (junction 2431) [order 2] : {
              | %Cound not found measurement twice,
              | % So not transfer tracker k to new list
              | }
          (junction 2432) -> (junction 2431)
          (junction 2433) -> (junction 2432)
          (junction 2434) -> (junction 2433)
          (junction 2431) -> (junction 2435) : {
              | Updatereturn=0;Ini_Tracker_UpdateFlg=0;
              | }
        state Ini_ThridTime_LR [function]
          (default) -> (junction 2461) : {
              | RelDeg=0;Min_Distance_IniTrack=9;RelativeDist=0;
              | x_3_predict=2*Ini_Tracker_LRSRR[k][6]-Ini_Tracker_LRSRR[k][4];%Use two point to predict next point based constant velocity
              | y_3_predict=2*Ini_Tracker_LRSRR[k][7]-Ini_Tracker_LRSRR[k][5];%Use two point to predict next point based constant velocity
              | Updatereturn=0;Ini_Tracker_UpdateFlg=0;
              | }
          (junction 2461) -> (junction 2910) [order 1] : [(j<Num_Returns)]
          (junction 2910) -> (junction 2462) [order 1] : [(Returns[j][2]==0)]
          (junction 2912) -> (junction 2461) : {
              | j++;
              | }
          (junction 2462) -> (junction 2463) : {
              | RelativeDist=(x_3_predict-Returns[j][0])*(x_3_predict-Returns[j][0])+(y_3_predict-Returns[j][1])*(y_3_predict-Returns[j][1]);
              | RelDeg=cos_cal(Ini_Tracker_LRSRR[k][4],Ini_Tracker_LRSRR[k][5],...
              | Ini_Tracker_LRSRR[k][6],Ini_Tracker_LRSRR[k][7],Returns[j][0],Returns[j][1]);
              | }
          (junction 2461) -> (junction 2469) [order 2] : {
              | j=0;
              | }
          (junction 2910) -> (junction 2912) [order 2]
          (junction 2463) -> (junction 3067) [order 1] : [(RelativeDist<4)]
          (junction 3067) -> (junction 3070) [order 1] : [(RelativeDist<0.1)]
          (junction 2463) -> (junction 2466) [order 2]
          (junction 3067) -> (junction 3071) [order 2]
          (junction 3070) -> (junction 3053)
          (junction 3071) -> (junction 3053) [order 1] : [(((RelDeg>120) || (RelDeg<60)))]
          (junction 3053) -> (junction 3057) [order 1] : [RelativeDist<Min_Distance_IniTrack]
          (junction 3071) -> (junction 3065) [order 2]
          (junction 3053) -> (junction 3061) [order 2]
          (junction 3057) -> (junction 3059) : {
              | Updatereturn=j;
              | Ini_Tracker_UpdateFlg=1;
              | Min_Distance_IniTrack=RelativeDist;
              | }
          (junction 2466) -> (junction 2912)
          (junction 3065) -> (junction 2466)
          (junction 3061) -> (junction 3065)
          (junction 3059) -> (junction 3061)
          (junction 2469) -> (junction 2470) [order 1] : [Ini_Tracker_UpdateFlg==1]%Means that the tracker k found measurement
          (junction 2469) -> (junction 2471) [order 2] : {
              | Ini_Tracker_LRSRR_New[Num_Ini_Tracker_LRSRR_New][0]=x_3_predict;
              | Ini_Tracker_LRSRR_New[Num_Ini_Tracker_LRSRR_New][1]=y_3_predict;
              | Ini_Tracker_LRSRR_New[Num_Ini_Tracker_LRSRR_New][2]=3;%Tracker counter
              | Ini_Tracker_LRSRR_New[Num_Ini_Tracker_LRSRR_New][3]=2;%Association counter
              | Ini_Tracker_LRSRR_New[Num_Ini_Tracker_LRSRR_New][4]=Ini_Tracker_LRSRR[k][4];
              | Ini_Tracker_LRSRR_New[Num_Ini_Tracker_LRSRR_New][5]=Ini_Tracker_LRSRR[k][5];
              | Ini_Tracker_LRSRR_New[Num_Ini_Tracker_LRSRR_New][6]=Ini_Tracker_LRSRR[k][6];
              | Ini_Tracker_LRSRR_New[Num_Ini_Tracker_LRSRR_New][7]=Ini_Tracker_LRSRR[k][7];
              | Ini_Tracker_LRSRR_New[Num_Ini_Tracker_LRSRR_New][8]=x_3_predict;
              | Ini_Tracker_LRSRR_New[Num_Ini_Tracker_LRSRR_New][9]=y_3_predict;
              | Num_Ini_Tracker_LRSRR_New++;
              | }
          (junction 2470) -> (junction 2472) : {
              | Returns[Updatereturn][2]=1;%Which means that the return is used
              | Ini_Tracker_LRSRR_New[Num_Ini_Tracker_LRSRR_New][0]=Returns[Updatereturn][0];
              | Ini_Tracker_LRSRR_New[Num_Ini_Tracker_LRSRR_New][1]=Returns[Updatereturn][1];
              | Ini_Tracker_LRSRR_New[Num_Ini_Tracker_LRSRR_New][2]=3;%Tracker counter
              | Ini_Tracker_LRSRR_New[Num_Ini_Tracker_LRSRR_New][3]=3;%Association counter
              | Ini_Tracker_LRSRR_New[Num_Ini_Tracker_LRSRR_New][4]=Ini_Tracker_LRSRR[k][4];
              | Ini_Tracker_LRSRR_New[Num_Ini_Tracker_LRSRR_New][5]=Ini_Tracker_LRSRR[k][5];
              | Ini_Tracker_LRSRR_New[Num_Ini_Tracker_LRSRR_New][6]=Ini_Tracker_LRSRR[k][6];
              | Ini_Tracker_LRSRR_New[Num_Ini_Tracker_LRSRR_New][7]=Ini_Tracker_LRSRR[k][7];
              | Ini_Tracker_LRSRR_New[Num_Ini_Tracker_LRSRR_New][8]=Returns[Updatereturn][0];
              | Ini_Tracker_LRSRR_New[Num_Ini_Tracker_LRSRR_New][9]=Returns[Updatereturn][1];
              | Num_Ini_Tracker_LRSRR_New++;
              | }
          (junction 2472) -> (junction 2471)
          (junction 2471) -> (junction 2473) : {
              | Updatereturn=0;Ini_Tracker_UpdateFlg=0;
              | }
        state Ini_SecondTime_LR [function]
          (default) -> (junction 2492) : {
              | AssoFlgtm=0;
              | }
          (junction 2492) -> (junction 2493) [order 1] : [j<Num_Returns]
          (junction 2494) -> (junction 2492) : {
              | j++;
              | }
          (junction 2493) -> (junction 2494) : {
              | AssoFlgtm[j]=VelocityMethod(Ini_Tracker_LRSRR[k][4],Ini_Tracker_LRSRR[k][5],...
              | Returns[j][0],Returns[j][1],10,0,5,0,1.5,1.5,5,0.04);%Velocity Association method
              | }
          (junction 2492) -> (junction 2495) [order 2] : {
              | j=0;
              | }
          (junction 2495) -> (junction 2496) [order 1] : [j<Num_Returns]
          (junction 2496) -> (junction 2497) [order 1] : [AssoFlgtm[j]==1]
          (junction 2499) -> (junction 2495) : {
              | j++;
              | }
          (junction 2495) -> (junction 2498) [order 2] : {
              | j=0;
              | AssoFlgtm=0;
              | }
          (junction 2496) -> (junction 2499) [order 2]
          (junction 2497) -> (junction 2500) : {
              | Returns[j][2]=1;%Which means that the return is used
              | Ini_Tracker_LRSRR_New[Num_Ini_Tracker_LRSRR_New][0]=Returns[j][0];
              | Ini_Tracker_LRSRR_New[Num_Ini_Tracker_LRSRR_New][1]=Returns[j][1];
              | Ini_Tracker_LRSRR_New[Num_Ini_Tracker_LRSRR_New][2]=2;
              | Ini_Tracker_LRSRR_New[Num_Ini_Tracker_LRSRR_New][3]=2;
              | Ini_Tracker_LRSRR_New[Num_Ini_Tracker_LRSRR_New][4]=Ini_Tracker_LRSRR[k][4];
              | Ini_Tracker_LRSRR_New[Num_Ini_Tracker_LRSRR_New][5]=Ini_Tracker_LRSRR[k][5];
              | Ini_Tracker_LRSRR_New[Num_Ini_Tracker_LRSRR_New][6]=Returns[j][0];
              | Ini_Tracker_LRSRR_New[Num_Ini_Tracker_LRSRR_New][7]=Returns[j][1];
              | Num_Ini_Tracker_LRSRR_New++;
              | }
          (junction 2500) -> (junction 2499)
        (default) -> (junction 2347)
        (junction 2347) -> (junction 2348) [order 1] : [Ini_Tracker_LRSRR[k][2]==4]%This Tracker has updated forth and find fifth measurement
        (junction 2347) -> (junction 2349) [order 2]
        (junction 2348) -> (junction 2350) : {
            | Ini_FifthTime_LR();
            | }
        (junction 2350) -> (junction 2349)
        (junction 2349) -> (junction 2351)
        (junction 2351) -> (junction 2352) [order 1] : [Ini_Tracker_LRSRR[k][2]==3]%This Tracker has updated thrid and find forth measurement
        (junction 2351) -> (junction 2353) [order 2]
        (junction 2352) -> (junction 2354) : {
            | Ini_ForthTime_LR();
            | }
        (junction 2354) -> (junction 2353)
        (junction 2353) -> (junction 2355)
        (junction 2355) -> (junction 2356) [order 1] : [Ini_Tracker_LRSRR[k][2]==2]%This Tracker has updated once and find thrid measurement
        (junction 2355) -> (junction 2357) [order 2]
        (junction 2356) -> (junction 2358) : {
            | Ini_ThridTime_LR();
            | }
        (junction 2358) -> (junction 2357)
        (junction 2357) -> (junction 2359)
        (junction 2359) -> (junction 2360) [order 1] : [Ini_Tracker_LRSRR[k][2]==1]%This Tracker is first initial and use velocity to find next measurements
        (junction 2359) -> (junction 2361) [order 2]
        (junction 2360) -> (junction 2362) : {
            | Ini_SecondTime_LR();
            | }
        (junction 2362) -> (junction 2361)
        (junction 2361) -> (junction 2363)
      state LRFirstTrackGen [function]
        (default) -> (junction 3438)
        (junction 3438) -> (junction 3439) [order 1] : [Num_Returns>1]%Two return, begine compare
        (junction 3438) -> (junction 3446) [order 2]
        (junction 3439) -> (junction 3445) : {
            | j=1;
            | }
        (junction 3440) -> (junction 3441) [order 1] : [(Returns[k][0]-Returns[j][0])*(Returns[k][0]-Returns[j][0])+...
            | (Returns[k][1]-Returns[j][1])*(Returns[k][1]-Returns[j][1])<=9]
        (junction 3444) -> (junction 3440) [order 1] : [Returns[j][2]==0]
        (junction 3442) -> (junction 3443) [order 1] : [Returns[k][2]==0]
        (junction 3443) -> (junction 3444) [order 1] : [j<Num_Returns]
        (junction 3445) -> (junction 3442) [order 1] : [k<Num_Returns-1]
        (junction 3448) -> (junction 3443) : {
            | j++;
            | }
        (junction 3440) -> (junction 3449) [order 2]
        (junction 3441) -> (junction 3450) : {
            | Group_Data[Group_Num][0]=Returns[j][0];
            | Group_Data[Group_Num][1]=Returns[j][1];
            | Returns[j][2]=1;
            | Group_Num=Group_Num+1;
            | }
        (junction 3451) -> (junction 3445) : {
            | k++;
            | j=k+1;
            | Group_Num=0;
            | Group_Data=0;
            | Group_X=0;
            | Group_Y=0;
            | }
        (junction 3442) -> (junction 3451) [order 2]
        (junction 3443) -> (junction 3452) [order 2] : {
            | Group_X=Returns[k][0];
            | Group_Y=Returns[k][1];
            | }
        (junction 3444) -> (junction 3448) [order 2]
        (junction 3445) -> (junction 3460) [order 2] : {
            | k=0;
            | j=0;
            | }
        (junction 3446) -> (junction 3447) [order 1] : [(Num_Returns==1) && (Returns[0][2]==0)]%One return, no need to compare
        (junction 3446) -> (junction 3458) [order 2]
        (junction 3447) -> (junction 3459) : {
            | Ini_Tracker_LRSRR_New[Num_Ini_Tracker_LRSRR_New][0]=Returns[0][0];
            | Ini_Tracker_LRSRR_New[Num_Ini_Tracker_LRSRR_New][1]=Returns[0][1];
            | Ini_Tracker_LRSRR_New[Num_Ini_Tracker_LRSRR_New][2]=1;
            | Ini_Tracker_LRSRR_New[Num_Ini_Tracker_LRSRR_New][3]=1;
            | Ini_Tracker_LRSRR_New[Num_Ini_Tracker_LRSRR_New][4]=Returns[0][0];
            | Ini_Tracker_LRSRR_New[Num_Ini_Tracker_LRSRR_New][5]=Returns[0][1];
            | Ini_Tracker_LRSRR_New[Num_Ini_Tracker_LRSRR_New][6]=0;
            | Ini_Tracker_LRSRR_New[Num_Ini_Tracker_LRSRR_New][7]=0;
            | Ini_Tracker_LRSRR_New[Num_Ini_Tracker_LRSRR_New][8]=0;
            | Ini_Tracker_LRSRR_New[Num_Ini_Tracker_LRSRR_New][9]=0;
            | Ini_Tracker_LRSRR_New[Num_Ini_Tracker_LRSRR_New][10]=0;
            | Ini_Tracker_LRSRR_New[Num_Ini_Tracker_LRSRR_New][11]=0;
            | Num_Ini_Tracker_LFSRR_New++;
            | }
        (junction 3449) -> (junction 3448)
        (junction 3450) -> (junction 3449)
        (junction 3452) -> (junction 3453) [order 1] : [Group_Num>0]%There exist more than one near unused returns
        (junction 3453) -> (junction 3454) [order 1] : [n<Group_Num]
        (junction 3455) -> (junction 3453) : {
            | n++;
            | }
        (junction 3461) -> (junction 3451)
        (junction 3452) -> (junction 3456) [order 2]
        (junction 3453) -> (junction 3457) [order 2] : {
            | n=0;
            | Group_X=Group_X/(Group_Num+1);Group_Y=Group_Y/(Group_Num+1);
            | }
        (junction 3454) -> (junction 3455) : {
            | Group_X=Group_X+Group_Data[n][0];
            | Group_Y=Group_Y+Group_Data[n][1];
            | }
        (junction 3457) -> (junction 3456)
        (junction 3456) -> (junction 3462) : {
            | Ini_Tracker_LRSRR_New[Num_Ini_Tracker_LRSRR_New][0]=Group_X;
            | Ini_Tracker_LRSRR_New[Num_Ini_Tracker_LRSRR_New][1]=Group_Y;
            | Ini_Tracker_LRSRR_New[Num_Ini_Tracker_LRSRR_New][2]=1;
            | Ini_Tracker_LRSRR_New[Num_Ini_Tracker_LRSRR_New][3]=1;
            | Ini_Tracker_LRSRR_New[Num_Ini_Tracker_LRSRR_New][4]=Group_X;
            | Ini_Tracker_LRSRR_New[Num_Ini_Tracker_LRSRR_New][5]=Group_Y;
            | Ini_Tracker_LRSRR_New[Num_Ini_Tracker_LRSRR_New][6]=0;
            | Ini_Tracker_LRSRR_New[Num_Ini_Tracker_LRSRR_New][7]=0;
            | Ini_Tracker_LRSRR_New[Num_Ini_Tracker_LRSRR_New][8]=0;
            | Ini_Tracker_LRSRR_New[Num_Ini_Tracker_LRSRR_New][9]=0;
            | Ini_Tracker_LRSRR_New[Num_Ini_Tracker_LRSRR_New][10]=0;
            | Ini_Tracker_LRSRR_New[Num_Ini_Tracker_LRSRR_New][11]=0;
            | Num_Ini_Tracker_LRSRR_New++;
            | }
        (junction 3459) -> (junction 3458)
        (junction 3460) -> (junction 3459)
        (junction 3462) -> (junction 3461)
        (junction 3458) -> (junction 3463)
      (default) -> (junction 2515) : {
          | Ini_Tracker_LRSRR=Ini_Tracker_LRSRR_New;
          | Num_Ini_Tracker_LRSRR=Num_Ini_Tracker_LRSRR_New;
          | Num_Ini_Tracker_LRSRR_New=0;Ini_Tracker_LRSRR_New=0;
          | AssoFlgtm=0;Group_Data=0;Group_Num=0;
          | }
      (junction 2515) -> (junction 2325) [order 1] : [k<30]
      (junction 2325) -> (junction 2320) [order 1] : [Ini_Tracker_LRSRR[k][2]>0]
      (junction 2514) -> (junction 2515) : {
          | k++;
          | }
      (junction 2515) -> (junction 2516) [order 2] : {
          | k=0;
          | }
      (junction 2325) -> (junction 2514) [order 2]
      (junction 2320) -> (junction 2343) : {
          | LRSRR_Ini_Update();
          | }
      (junction 2343) -> (junction 2514)
      (junction 2516) -> (junction 2322) : {
          | LRFirstTrackGen();
          | }
    state RRSRR_Ini [function]
      state RRSRR_Ini_Update [function]
        note: %Recently used in 4/5 logical modle in the initial of radar tracker
        state Ini_FifthTime_RR [function]
          (default) -> (junction 2566) : {
              | RelDeg=0;Min_Distance_IniTrack=9;RelativeDist=0;
              | x_5_predict=3*Ini_Tracker_RRSRR[k][10]-3*Ini_Tracker_RRSRR[k][8]+Ini_Tracker_RRSRR[k][6];%Use three point to predict next point based constant acc
              | y_5_predict=3*Ini_Tracker_RRSRR[k][11]-3*Ini_Tracker_RRSRR[k][9]+Ini_Tracker_RRSRR[k][7];%Use three point to predict next point based constant acc
              | Updatereturn=0;Ini_Tracker_UpdateFlg=0;
              | }
          (junction 2566) -> (junction 2935) [order 1] : [(j<Num_Returns)]
          (junction 2935) -> (junction 2567) [order 1] : [(Returns[j][2]==0)]
          (junction 2937) -> (junction 2566) : {
              | j++;
              | }
          (junction 2567) -> (junction 2568) : {
              | RelativeDist=(x_5_predict-Returns[j][0])*(x_5_predict-Returns[j][0])+(y_5_predict-Returns[j][1])*(y_5_predict-Returns[j][1]);
              | RelDeg=cos_cal(Ini_Tracker_RRSRR[k][8],Ini_Tracker_RRSRR[k][9],...
              | Ini_Tracker_RRSRR[k][10],Ini_Tracker_RRSRR[k][11],Returns[j][0],Returns[j][1]);
              | }
          (junction 2566) -> (junction 2574) [order 2] : {
              | j=0;
              | }
          (junction 2935) -> (junction 2937) [order 2]
          (junction 2568) -> (junction 3167) [order 1] : [(RelativeDist<4)]
          (junction 3167) -> (junction 3170) [order 1] : [(RelativeDist<0.1)]
          (junction 2568) -> (junction 2571) [order 2]
          (junction 3167) -> (junction 3171) [order 2]
          (junction 3170) -> (junction 3153)
          (junction 3171) -> (junction 3153) [order 1] : [(((RelDeg>120) || (RelDeg<60)))]
          (junction 3153) -> (junction 3157) [order 1] : [RelativeDist<Min_Distance_IniTrack]
          (junction 3171) -> (junction 3165) [order 2]
          (junction 3153) -> (junction 3161) [order 2]
          (junction 3157) -> (junction 3159) : {
              | Updatereturn=j;
              | Ini_Tracker_UpdateFlg=1;
              | Min_Distance_IniTrack=RelativeDist;
              | }
          (junction 2571) -> (junction 2937)
          (junction 3165) -> (junction 2571)
          (junction 3161) -> (junction 3165)
          (junction 3159) -> (junction 3161)
          (junction 2574) -> (junction 2575) [order 1] : [Ini_Tracker_UpdateFlg==1]%Means that the tracker k found measurement
          (junction 2574) -> (junction 2576) [order 2] : {
              | %cound not found, and enter 5 searches means that could not found once before, so delete
              | }
          (junction 2575) -> (junction 2577) : {
              | Returns[Updatereturn][2]=1;
              | %Which means that the return is used
              | TrackIni(Returns[Updatereturn][0],Returns[Updatereturn][1]);
              | }
          (junction 2577) -> (junction 2576)
          (junction 2576) -> (junction 2578) : {
              | Updatereturn=0;Ini_Tracker_UpdateFlg=0;
              | }
        state Ini_ForthTime_RR [function]
          (default) -> (junction 2597) : {
              | RelDeg=0;Min_Distance_IniTrack=9;RelativeDist=0;
              | x_4_predict=3*Ini_Tracker_RRSRR[k][8]-3*Ini_Tracker_RRSRR[k][6]+Ini_Tracker_RRSRR[k][4];%Use three point to predict next point based constant acc
              | y_4_predict=3*Ini_Tracker_RRSRR[k][9]-3*Ini_Tracker_RRSRR[k][7]+Ini_Tracker_RRSRR[k][5];%Use three point to predict next point based constant acc
              | Updatereturn=0;Ini_Tracker_UpdateFlg=0;
              | }
          (junction 2597) -> (junction 2930) [order 1] : [(j<Num_Returns) ]
          (junction 2930) -> (junction 2598) [order 1] : [(Returns[j][2]==0)]
          (junction 2932) -> (junction 2597) : {
              | j++;
              | }
          (junction 2597) -> (junction 2605) [order 2] : {
              | j=0;
              | }
          (junction 2930) -> (junction 2932) [order 2]
          (junction 2598) -> (junction 2599) : {
              | RelativeDist=(x_4_predict-Returns[j][0])*(x_4_predict-Returns[j][0])+(y_4_predict-Returns[j][1])*(y_4_predict-Returns[j][1]);
              | RelDeg=cos_cal(Ini_Tracker_RRSRR[k][6],Ini_Tracker_RRSRR[k][7],...
              | Ini_Tracker_RRSRR[k][8],Ini_Tracker_RRSRR[k][9],Returns[j][0],Returns[j][1]);
              | }
          (junction 2599) -> (junction 3147) [order 1] : [(RelativeDist<4)]
          (junction 3147) -> (junction 3150) [order 1] : [(RelativeDist<0.1)]
          (junction 2599) -> (junction 2602) [order 2]
          (junction 3147) -> (junction 3151) [order 2]
          (junction 3150) -> (junction 3133)
          (junction 3151) -> (junction 3133) [order 1] : [(((RelDeg>120) || (RelDeg<60)))]
          (junction 3133) -> (junction 3137) [order 1] : [RelativeDist<Min_Distance_IniTrack]
          (junction 3151) -> (junction 3145) [order 2]
          (junction 3133) -> (junction 3141) [order 2]
          (junction 3137) -> (junction 3139) : {
              | Updatereturn=j;
              | Ini_Tracker_UpdateFlg=1;
              | Min_Distance_IniTrack=RelativeDist;
              | }
          (junction 2602) -> (junction 2932)
          (junction 3145) -> (junction 2602)
          (junction 3141) -> (junction 3145)
          (junction 3139) -> (junction 3141)
          (junction 2605) -> (junction 2606) [order 1] : [Ini_Tracker_UpdateFlg==1]%Means that the tracker k found measurement
          (junction 2606) -> (junction 2607) [order 1] : [Ini_Tracker_RRSRR[k][3]==3]%Has found measurement 4 times and begin ini
          (junction 2605) -> (junction 2609) [order 2]
          (junction 2606) -> (junction 2612) [order 2] : {
              | Returns[Updatereturn][2]=1;%Which means that the return is used
              | Ini_Tracker_LRSRR_New[Num_Ini_Tracker_RRSRR_New][0]=Returns[Updatereturn][0];
              | Ini_Tracker_LRSRR_New[Num_Ini_Tracker_RRSRR_New][1]=Returns[Updatereturn][1];
              | Ini_Tracker_LRSRR_New[Num_Ini_Tracker_RRSRR_New][2]=4;%Tracker counter
              | Ini_Tracker_LRSRR_New[Num_Ini_Tracker_RRSRR_New][3]=3;%Association counter
              | Ini_Tracker_LRSRR_New[Num_Ini_Tracker_RRSRR_New][4]=Ini_Tracker_RRSRR[k][4];
              | Ini_Tracker_LRSRR_New[Num_Ini_Tracker_RRSRR_New][5]=Ini_Tracker_RRSRR[k][5];
              | Ini_Tracker_LRSRR_New[Num_Ini_Tracker_RRSRR_New][6]=Ini_Tracker_RRSRR[k][6];
              | Ini_Tracker_LRSRR_New[Num_Ini_Tracker_RRSRR_New][7]=Ini_Tracker_RRSRR[k][7];
              | Ini_Tracker_LRSRR_New[Num_Ini_Tracker_RRSRR_New][8]=Ini_Tracker_RRSRR[k][8];
              | Ini_Tracker_LRSRR_New[Num_Ini_Tracker_RRSRR_New][9]=Ini_Tracker_RRSRR[k][9];
              | Ini_Tracker_LRSRR_New[Num_Ini_Tracker_RRSRR_New][10]=Returns[Updatereturn][0];
              | Ini_Tracker_LRSRR_New[Num_Ini_Tracker_RRSRR_New][11]=Returns[Updatereturn][1];
              | Num_Ini_Tracker_RRSRR_New++;
              | }
          (junction 2607) -> (junction 2613) : {
              | Returns[Updatereturn][2]=1;
              | %Which means that the return is used
              | TrackIni(Returns[Updatereturn][0],Returns[Updatereturn][1]);
              | }
          (junction 2609) -> (junction 2608) [order 1] : [Ini_Tracker_RRSRR[k][3]==3]
              | %Has found measurement 3 times before
          (junction 2608) -> (junction 2611) : {
              | Ini_Tracker_RRSRR_New[Num_Ini_Tracker_RRSRR_New][0]=x_4_predict;
              | Ini_Tracker_RRSRR_New[Num_Ini_Tracker_RRSRR_New][1]=y_4_predict;
              | Ini_Tracker_RRSRR_New[Num_Ini_Tracker_RRSRR_New][2]=4;%Tracker counter
              | Ini_Tracker_RRSRR_New[Num_Ini_Tracker_RRSRR_New][3]=3;%Association counter
              | Ini_Tracker_RRSRR_New[Num_Ini_Tracker_RRSRR_New][4]=Ini_Tracker_RRSRR[k][4];
              | Ini_Tracker_RRSRR_New[Num_Ini_Tracker_RRSRR_New][5]=Ini_Tracker_RRSRR[k][5];
              | Ini_Tracker_RRSRR_New[Num_Ini_Tracker_RRSRR_New][6]=Ini_Tracker_RRSRR[k][6];
              | Ini_Tracker_RRSRR_New[Num_Ini_Tracker_RRSRR_New][7]=Ini_Tracker_RRSRR[k][7];
              | Ini_Tracker_RRSRR_New[Num_Ini_Tracker_RRSRR_New][8]=Ini_Tracker_RRSRR[k][8];
              | Ini_Tracker_RRSRR_New[Num_Ini_Tracker_RRSRR_New][9]=Ini_Tracker_RRSRR[k][9];
              | Ini_Tracker_RRSRR_New[Num_Ini_Tracker_RRSRR_New][10]=x_4_predict;
              | Ini_Tracker_RRSRR_New[Num_Ini_Tracker_RRSRR_New][11]=y_4_predict;
              | Num_Ini_Tracker_RRSRR_New++;
              | }
          (junction 2609) -> (junction 2610) [order 2] : {
              | %Cound not found measurement twice,
              | % So not transfer tracker k to new list
              | }
          (junction 2611) -> (junction 2610)
          (junction 2612) -> (junction 2611)
          (junction 2613) -> (junction 2612)
          (junction 2610) -> (junction 2614) : {
              | Updatereturn=0;Ini_Tracker_UpdateFlg=0;
              | }
        state Ini_ThridTime_RR [function]
          (default) -> (junction 2640) : {
              | RelDeg=0;Min_Distance_IniTrack=9;RelativeDist=0;
              | x_3_predict=2*Ini_Tracker_RRSRR[k][6]-Ini_Tracker_RRSRR[k][4];%Use two point to predict next point based constant velocity
              | y_3_predict=2*Ini_Tracker_RRSRR[k][7]-Ini_Tracker_RRSRR[k][5];%Use two point to predict next point based constant velocity
              | Updatereturn=0;Ini_Tracker_UpdateFlg=0;
              | }
          (junction 2640) -> (junction 2925) [order 1] : [(j<Num_Returns)]
          (junction 2925) -> (junction 2641) [order 1] : [(Returns[j][2]==0)]
          (junction 2927) -> (junction 2640) : {
              | j++;
              | }
          (junction 2640) -> (junction 2648) [order 2] : {
              | j=0;
              | }
          (junction 2925) -> (junction 2927) [order 2]
          (junction 2641) -> (junction 2642) : {
              | RelativeDist=(x_3_predict-Returns[j][0])*(x_3_predict-Returns[j][0])+(y_3_predict-Returns[j][1])*(y_3_predict-Returns[j][1]);
              | RelDeg=cos_cal(Ini_Tracker_LRSRR[k][4],Ini_Tracker_RRSRR[k][5],...
              | Ini_Tracker_RRSRR[k][6],Ini_Tracker_RRSRR[k][7],Returns[j][0],Returns[j][1]);
              | }
          (junction 2642) -> (junction 3127) [order 1] : [(RelativeDist<4)]
          (junction 3127) -> (junction 3130) [order 1] : [(RelativeDist<0.1)]
          (junction 2642) -> (junction 2645) [order 2]
          (junction 3127) -> (junction 3131) [order 2]
          (junction 3130) -> (junction 3113)
          (junction 3131) -> (junction 3113) [order 1] : [(((RelDeg>120) || (RelDeg<60)))]
          (junction 3113) -> (junction 3117) [order 1] : [RelativeDist<Min_Distance_IniTrack]
          (junction 3131) -> (junction 3125) [order 2]
          (junction 3113) -> (junction 3121) [order 2]
          (junction 3117) -> (junction 3119) : {
              | Updatereturn=j;
              | Ini_Tracker_UpdateFlg=1;
              | Min_Distance_IniTrack=RelativeDist;
              | }
          (junction 2645) -> (junction 2927)
          (junction 3125) -> (junction 2645)
          (junction 3121) -> (junction 3125)
          (junction 3119) -> (junction 3121)
          (junction 2648) -> (junction 2649) [order 1] : [Ini_Tracker_UpdateFlg==1]%Means that the tracker k found measurement
          (junction 2648) -> (junction 2650) [order 2] : {
              | Ini_Tracker_RRSRR_New[Num_Ini_Tracker_RRSRR_New][0]=x_3_predict;
              | Ini_Tracker_RRSRR_New[Num_Ini_Tracker_RRSRR_New][1]=y_3_predict;
              | Ini_Tracker_RRSRR_New[Num_Ini_Tracker_RRSRR_New][2]=3;%Tracker counter
              | Ini_Tracker_RRSRR_New[Num_Ini_Tracker_RRSRR_New][3]=2;%Association counter
              | Ini_Tracker_RRSRR_New[Num_Ini_Tracker_RRSRR_New][4]=Ini_Tracker_RRSRR[k][4];
              | Ini_Tracker_RRSRR_New[Num_Ini_Tracker_RRSRR_New][5]=Ini_Tracker_RRSRR[k][5];
              | Ini_Tracker_RRSRR_New[Num_Ini_Tracker_RRSRR_New][6]=Ini_Tracker_RRSRR[k][6];
              | Ini_Tracker_RRSRR_New[Num_Ini_Tracker_RRSRR_New][7]=Ini_Tracker_RRSRR[k][7];
              | Ini_Tracker_RRSRR_New[Num_Ini_Tracker_RRSRR_New][8]=x_3_predict;
              | Ini_Tracker_RRSRR_New[Num_Ini_Tracker_RRSRR_New][9]=y_3_predict;
              | Num_Ini_Tracker_RRSRR_New++;
              | }
          (junction 2649) -> (junction 2651) : {
              | Returns[Updatereturn][2]=1;%Which means that the return is used
              | Ini_Tracker_RRSRR_New[Num_Ini_Tracker_RRSRR_New][0]=Returns[Updatereturn][0];
              | Ini_Tracker_RRSRR_New[Num_Ini_Tracker_RRSRR_New][1]=Returns[Updatereturn][1];
              | Ini_Tracker_RRSRR_New[Num_Ini_Tracker_RRSRR_New][2]=3;%Tracker counter
              | Ini_Tracker_RRSRR_New[Num_Ini_Tracker_RRSRR_New][3]=3;%Association counter
              | Ini_Tracker_RRSRR_New[Num_Ini_Tracker_RRSRR_New][4]=Ini_Tracker_RRSRR[k][4];
              | Ini_Tracker_RRSRR_New[Num_Ini_Tracker_RRSRR_New][5]=Ini_Tracker_RRSRR[k][5];
              | Ini_Tracker_RRSRR_New[Num_Ini_Tracker_RRSRR_New][6]=Ini_Tracker_RRSRR[k][6];
              | Ini_Tracker_RRSRR_New[Num_Ini_Tracker_RRSRR_New][7]=Ini_Tracker_RRSRR[k][7];
              | Ini_Tracker_RRSRR_New[Num_Ini_Tracker_RRSRR_New][8]=Returns[Updatereturn][0];
              | Ini_Tracker_RRSRR_New[Num_Ini_Tracker_RRSRR_New][9]=Returns[Updatereturn][1];
              | Num_Ini_Tracker_RRSRR_New++;
              | }
          (junction 2651) -> (junction 2650)
          (junction 2650) -> (junction 2652) : {
              | Updatereturn=0;Ini_Tracker_UpdateFlg=0;
              | }
        state Ini_SecondTime_RR [function]
          (default) -> (junction 2671) : {
              | AssoFlgtm=0;
              | }
          (junction 2671) -> (junction 2672) [order 1] : [j<Num_Returns]
          (junction 2673) -> (junction 2671) : {
              | j++;
              | }
          (junction 2672) -> (junction 2673) : {
              | AssoFlgtm[j]=VelocityMethod(Ini_Tracker_RRSRR[k][4],Ini_Tracker_RRSRR[k][5],...
              | Returns[j][0],Returns[j][1],10,0,5,0,1.5,1.5,5,0.04);%Velocity Association method
              | }
          (junction 2671) -> (junction 2674) [order 2] : {
              | j=0;
              | }
          (junction 2674) -> (junction 2675) [order 1] : [j<Num_Returns]
          (junction 2675) -> (junction 2676) [order 1] : [AssoFlgtm[j]==1]
          (junction 2678) -> (junction 2674) : {
              | j++;
              | }
          (junction 2674) -> (junction 2677) [order 2] : {
              | j=0;
              | AssoFlgtm=0;
              | }
          (junction 2675) -> (junction 2678) [order 2]
          (junction 2676) -> (junction 2679) : {
              | Returns[j][2]=1;%Which means that the return is used
              | Ini_Tracker_RRSRR_New[Num_Ini_Tracker_RRSRR_New][0]=Returns[j][0];
              | Ini_Tracker_RRSRR_New[Num_Ini_Tracker_RRSRR_New][1]=Returns[j][1];
              | Ini_Tracker_RRSRR_New[Num_Ini_Tracker_RRSRR_New][2]=2;
              | Ini_Tracker_RRSRR_New[Num_Ini_Tracker_RRSRR_New][3]=2;
              | Ini_Tracker_RRSRR_New[Num_Ini_Tracker_RRSRR_New][4]=Ini_Tracker_RRSRR[k][4];
              | Ini_Tracker_RRSRR_New[Num_Ini_Tracker_RRSRR_New][5]=Ini_Tracker_RRSRR[k][5];
              | Ini_Tracker_RRSRR_New[Num_Ini_Tracker_RRSRR_New][6]=Returns[j][0];
              | Ini_Tracker_RRSRR_New[Num_Ini_Tracker_RRSRR_New][7]=Returns[j][1];
              | Num_Ini_Tracker_RRSRR_New++;
              | }
          (junction 2679) -> (junction 2678)
        (default) -> (junction 2526)
        (junction 2526) -> (junction 2527) [order 1] : [Ini_Tracker_RRSRR[k][2]==4]%This Tracker has updated forth and find fifth measurement
        (junction 2526) -> (junction 2528) [order 2]
        (junction 2527) -> (junction 2529) : {
            | Ini_FifthTime_RR();
            | }
        (junction 2529) -> (junction 2528)
        (junction 2528) -> (junction 2530)
        (junction 2530) -> (junction 2531) [order 1] : [Ini_Tracker_RRSRR[k][2]==3]%This Tracker has updated thrid and find forth measurement
        (junction 2530) -> (junction 2532) [order 2]
        (junction 2531) -> (junction 2533) : {
            | Ini_ForthTime_RR();
            | }
        (junction 2533) -> (junction 2532)
        (junction 2532) -> (junction 2534)
        (junction 2534) -> (junction 2535) [order 1] : [Ini_Tracker_RRSRR[k][2]==2]%This Tracker has updated once and find thrid measurement
        (junction 2534) -> (junction 2536) [order 2]
        (junction 2535) -> (junction 2537) : {
            | Ini_ThridTime_RR();
            | }
        (junction 2537) -> (junction 2536)
        (junction 2536) -> (junction 2538)
        (junction 2538) -> (junction 2539) [order 1] : [Ini_Tracker_RRSRR[k][2]==1]%This Tracker is first initial and use velocity to find next measurements
        (junction 2538) -> (junction 2540) [order 2]
        (junction 2539) -> (junction 2541) : {
            | Ini_SecondTime_RR();
            | }
        (junction 2541) -> (junction 2540)
        (junction 2540) -> (junction 2542)
      state RRFirstTrackGen [function]
        (default) -> (junction 3500)
        (junction 3500) -> (junction 3501) [order 1] : [Num_Returns>1]%Two return, begine compare
        (junction 3500) -> (junction 3508) [order 2]
        (junction 3501) -> (junction 3507) : {
            | j=1;
            | }
        (junction 3502) -> (junction 3503) [order 1] : [(Returns[k][0]-Returns[j][0])*(Returns[k][0]-Returns[j][0])+...
            | (Returns[k][1]-Returns[j][1])*(Returns[k][1]-Returns[j][1])<=9]
        (junction 3506) -> (junction 3502) [order 1] : [Returns[j][2]==0]
        (junction 3504) -> (junction 3505) [order 1] : [Returns[k][2]==0]
        (junction 3505) -> (junction 3506) [order 1] : [j<Num_Returns]
        (junction 3507) -> (junction 3504) [order 1] : [k<Num_Returns-1]
        (junction 3510) -> (junction 3505) : {
            | j++;
            | }
        (junction 3502) -> (junction 3511) [order 2]
        (junction 3503) -> (junction 3512) : {
            | Group_Data[Group_Num][0]=Returns[j][0];
            | Group_Data[Group_Num][1]=Returns[j][1];
            | Returns[j][2]=1;
            | Group_Num=Group_Num+1;
            | }
        (junction 3513) -> (junction 3507) : {
            | k++;
            | j=k+1;
            | Group_Num=0;
            | Group_Data=0;
            | Group_X=0;
            | Group_Y=0;
            | }
        (junction 3504) -> (junction 3513) [order 2]
        (junction 3505) -> (junction 3514) [order 2] : {
            | Group_X=Returns[k][0];
            | Group_Y=Returns[k][1];
            | }
        (junction 3506) -> (junction 3510) [order 2]
        (junction 3507) -> (junction 3522) [order 2] : {
            | k=0;
            | j=0;
            | }
        (junction 3508) -> (junction 3509) [order 1] : [(Num_Returns==1) && (Returns[0][2]==0)]%One return, no need to compare
        (junction 3508) -> (junction 3520) [order 2]
        (junction 3509) -> (junction 3521) : {
            | Ini_Tracker_RRSRR_New[Num_Ini_Tracker_RRSRR_New][0]=Returns[0][0];
            | Ini_Tracker_RRSRR_New[Num_Ini_Tracker_RRSRR_New][1]=Returns[0][1];
            | Ini_Tracker_RRSRR_New[Num_Ini_Tracker_RRSRR_New][2]=1;
            | Ini_Tracker_RRSRR_New[Num_Ini_Tracker_RRSRR_New][3]=1;
            | Ini_Tracker_RRSRR_New[Num_Ini_Tracker_RRSRR_New][4]=Returns[0][0];
            | Ini_Tracker_RRSRR_New[Num_Ini_Tracker_RRSRR_New][5]=Returns[0][1];
            | Ini_Tracker_RRSRR_New[Num_Ini_Tracker_RRSRR_New][6]=0;
            | Ini_Tracker_RRSRR_New[Num_Ini_Tracker_RRSRR_New][7]=0;
            | Ini_Tracker_RRSRR_New[Num_Ini_Tracker_RRSRR_New][8]=0;
            | Ini_Tracker_RRSRR_New[Num_Ini_Tracker_RRSRR_New][9]=0;
            | Ini_Tracker_RRSRR_New[Num_Ini_Tracker_RRSRR_New][10]=0;
            | Ini_Tracker_RRSRR_New[Num_Ini_Tracker_RRSRR_New][11]=0;
            | Num_Ini_Tracker_RRSRR_New++;
            | }
        (junction 3511) -> (junction 3510)
        (junction 3512) -> (junction 3511)
        (junction 3514) -> (junction 3515) [order 1] : [Group_Num>0]%There exist more than one near unused returns
        (junction 3515) -> (junction 3516) [order 1] : [n<Group_Num]
        (junction 3517) -> (junction 3515) : {
            | n++;
            | }
        (junction 3523) -> (junction 3513)
        (junction 3514) -> (junction 3518) [order 2]
        (junction 3515) -> (junction 3519) [order 2] : {
            | n=0;
            | Group_X=Group_X/(Group_Num+1);Group_Y=Group_Y/(Group_Num+1);
            | }
        (junction 3516) -> (junction 3517) : {
            | Group_X=Group_X+Group_Data[n][0];
            | Group_Y=Group_Y+Group_Data[n][1];
            | }
        (junction 3519) -> (junction 3518)
        (junction 3518) -> (junction 3524) : {
            | Ini_Tracker_RRSRR_New[Num_Ini_Tracker_RRSRR_New][0]=Group_X;
            | Ini_Tracker_RRSRR_New[Num_Ini_Tracker_RRSRR_New][1]=Group_Y;
            | Ini_Tracker_RRSRR_New[Num_Ini_Tracker_RRSRR_New][2]=1;
            | Ini_Tracker_RRSRR_New[Num_Ini_Tracker_RRSRR_New][3]=1;
            | Ini_Tracker_RRSRR_New[Num_Ini_Tracker_RRSRR_New][4]=Group_X;
            | Ini_Tracker_RRSRR_New[Num_Ini_Tracker_RRSRR_New][5]=Group_Y;
            | Ini_Tracker_RRSRR_New[Num_Ini_Tracker_RRSRR_New][6]=0;
            | Ini_Tracker_RRSRR_New[Num_Ini_Tracker_RRSRR_New][7]=0;
            | Ini_Tracker_RRSRR_New[Num_Ini_Tracker_RRSRR_New][8]=0;
            | Ini_Tracker_RRSRR_New[Num_Ini_Tracker_RRSRR_New][9]=0;
            | Ini_Tracker_RRSRR_New[Num_Ini_Tracker_RRSRR_New][10]=0;
            | Ini_Tracker_RRSRR_New[Num_Ini_Tracker_RRSRR_New][11]=0;
            | Num_Ini_Tracker_RRSRR_New++;
            | }
        (junction 3521) -> (junction 3520)
        (junction 3522) -> (junction 3521)
        (junction 3524) -> (junction 3523)
        (junction 3520) -> (junction 3525)
      (default) -> (junction 2517) : {
          | Ini_Tracker_RRSRR=Ini_Tracker_RRSRR_New;
          | Num_Ini_Tracker_RRSRR=Num_Ini_Tracker_RRSRR_New;
          | Num_Ini_Tracker_RRSRR_New=0;Ini_Tracker_RRSRR_New=0;
          | AssoFlgtm=0;Group_Data=0;Group_Num=0;
          | }
      (junction 2517) -> (junction 2696) [order 1] : [k<30]
      (junction 2696) -> (junction 2692) [order 1] : [Ini_Tracker_RRSRR[k][2]>0]
      (junction 2524) -> (junction 2517) : {
          | k++;
          | }
      (junction 2517) -> (junction 2518) [order 2] : {
          | k=0;
          | }
      (junction 2696) -> (junction 2524) [order 2]
      (junction 2692) -> (junction 2519) : {
          | RRSRR_Ini_Update();
          | }
      (junction 2519) -> (junction 2524)
      (junction 2518) -> (junction 2694) : {
          | RRFirstTrackGen();
          | }
    state AssociationFlag  = VelocityMethod(x_t,y_t,x_m,y_m,vx_max,vx_min,... [function]
      vy_max,vy_min,Rxx,Ryy,threshod,ts)
    state relative_degree  =  cos_cal(x1,y1,x2,y2,xm,ym) [function]
    state TrackIni(ini_x,ini_y) [function]
      (default) -> (junction 2716) : {
          | LoopError=0;
          | }
      (junction 2720) -> (junction 2721) : {LastFusID++;}
      (junction 2721) -> (junction 2722) [order 1] : [LastFusID<127]
      (junction 2716) -> (junction 2720) [order 1]
      (junction 2727) -> (junction 2720) : {
          | LoopError++;
          | }
      (junction 2721) -> (junction 2723) [order 2] : {LastFusID=1;}
      (junction 2722) -> (junction 2724)
      (junction 2716) -> (junction 2733) [order 2]
      (junction 2723) -> (junction 2724)
      (junction 2724) -> (junction 2728)
      (junction 2728) -> (junction 2727) [order 2] : [LoopError<126 && (IDUsedFlag[LastFusID]==1)]
      (junction 2728) -> (junction 2729) [order 1] : [IDUsedFlag[LastFusID]==0]
      (junction 2728) -> (junction 2736) [order 3]
      (junction 2729) -> (junction 2737) : {
          | IDUsedFlag[LastFusID]=1;
          | FusDataInternal_temp[TrackCounter][0]=LastFusID;FusDataInternal_temp[TrackCounter][1]=ini_x;
          | FusDataInternal_temp[TrackCounter][2]=0;FusDataInternal_temp[TrackCounter][3]=ini_y;
          | FusDataInternal_temp[TrackCounter][4]=0;FusDataInternal_temp[TrackCounter][5]=0;
          | FusDataInternal_temp[TrackCounter][6]=0;FusDataInternal_temp[TrackCounter][7]=2;
          | FusDataInternal_temp[TrackCounter][8]=0;FusDataInternal_temp[TrackCounter][9]=0;
          | FusDataInternal_temp[TrackCounter][10]=0;FusDataInternal_temp[TrackCounter][11]=0;
          | FusDataInternal_temp[TrackCounter][12]=2;FusDataInternal_temp[TrackCounter][13]=0;
          | FusDataInternal_temp[TrackCounter][14]=0;FusDataInternal_temp[TrackCounter][15]=0;
          | FusDataInternal_temp[TrackCounter][16]=0;FusDataInternal_temp[TrackCounter][17]=2;
          | FusDataInternal_temp[TrackCounter][18]=0;FusDataInternal_temp[TrackCounter][19]=0;
          | FusDataInternal_temp[TrackCounter][20]=0;FusDataInternal_temp[TrackCounter][21]=0;
          | FusDataInternal_temp[TrackCounter][22]=2;
          | FusDataInternal_temp[TrackCounter][23]=5;%FusMark
          | FusDataInternal_temp[TrackCounter][24]=0;%Confrimed Flag
          | TrackCounter++;
          | }
      (junction 2736) -> (junction 2733)
      (junction 2737) -> (junction 2736)
      (junction 2733) -> (junction 2785)
    (default) -> (junction 1486) : {
        | Unused_Return_Gen();%Select Unused returns for Tracker initial
        | }
    (junction 1486) -> (junction 1676) [order 1] : [DataSource==1]
    (junction 1486) -> (junction 1488) [order 2]
    (junction 1676) -> (junction 1678) : {
        | LFSRR_Ini();
        | }
    (junction 1678) -> (junction 1488)
    (junction 1488) -> (junction 1696)
    (junction 1696) -> (junction 1698) [order 1] : [DataSource==2]
    (junction 1696) -> (junction 1702) [order 2]
    (junction 1698) -> (junction 1700) : {
        | RFSRR_Ini();
        | }
    (junction 1700) -> (junction 1702)
    (junction 1702) -> (junction 1714)
    (junction 1714) -> (junction 1709) [order 1] : [DataSource==3]
    (junction 1714) -> (junction 1712) [order 2]
    (junction 1709) -> (junction 1713) : {
        | LRSRR_Ini();
        | }
    (junction 1713) -> (junction 1712)
    (junction 1712) -> (junction 1718)
    (junction 1718) -> (junction 1719) [order 1] : [DataSource==4]
    (junction 1718) -> (junction 1720) [order 2]
    (junction 1719) -> (junction 1723) : {
        | RRSRR_Ini();
        | }
    (junction 1723) -> (junction 1720)
    (junction 1720) -> (junction 1725)
  state Measurement_Gen [function]
    (default) -> (junction 261) : {
        | FusDataInternal_temp=0;
        | k=0;%Description: This model is used for generated measurement and the number of measurement [ID, X, Y, MoveInfo]
        | }
    (junction 1329) -> (junction 1319) [order 1] : [k<10]
    (junction 1319) -> (junction 1327) [order 1] : [LFSRR_Input[k][0] !=0]
    (junction 261) -> (junction 1329) [order 1] : [DataSource==1]
    (junction 1320) -> (junction 1329) : {
        | k++;
        | }
    (junction 1329) -> (junction 1331) [order 2]
    (junction 1319) -> (junction 1320) [order 2]
    (junction 1327) -> (junction 1321) : {
        | Measure_Data[Measure_Num][0]=LFSRR_Input[k][0];
        | Measure_Data[Measure_Num][1]=LFSRR_Input[k][1];
        | Measure_Data[Measure_Num][2]=LFSRR_Input[k][2];
        | Measure_Data[Measure_Num][3]=LFSRR_Input[k][3];
        | Measure_Num++;
        | }
    (junction 261) -> (junction 1333) [order 2]
    (junction 1321) -> (junction 1320)
    (junction 1331) -> (junction 1333)
    (junction 1333) -> (junction 292) : {
        | k=0;
        | }
    (junction 292) -> (junction 1348) [order 1] : [DataSource==2]
    (junction 1348) -> (junction 1339) [order 1] : [k<10]
    (junction 1339) -> (junction 1338) [order 1] : [RFSRR_Input[k][0] !=0]
    (junction 1336) -> (junction 1348) : {
        | k++;
        | }
    (junction 292) -> (junction 1351) [order 2]
    (junction 1348) -> (junction 1349) [order 2]
    (junction 1339) -> (junction 1336) [order 2]
    (junction 1338) -> (junction 1337) : {
        | Measure_Data[Measure_Num][0]=RFSRR_Input[k][0];
        | Measure_Data[Measure_Num][1]=RFSRR_Input[k][1];
        | Measure_Data[Measure_Num][2]=RFSRR_Input[k][2];
        | Measure_Data[Measure_Num][3]=RFSRR_Input[k][3];
        | Measure_Num++;
        | }
    (junction 1349) -> (junction 1351)
    (junction 1337) -> (junction 1336)
    (junction 1351) -> (junction 300) : {
        | k=0;
        | }
    (junction 300) -> (junction 1366) [order 1] : [DataSource==3]
    (junction 1366) -> (junction 1354) [order 1] : [k<10]
    (junction 1354) -> (junction 1356) [order 1] : [LRSRR_Input[k][0] !=0]
    (junction 1352) -> (junction 1366) : {
        | k++;
        | }
    (junction 300) -> (junction 1368) [order 2]
    (junction 1366) -> (junction 1367) [order 2]
    (junction 1354) -> (junction 1352) [order 2]
    (junction 1356) -> (junction 1353) : {
        | Measure_Data[Measure_Num][0]=LRSRR_Input[k][0];
        | Measure_Data[Measure_Num][1]=LRSRR_Input[k][1];
        | Measure_Data[Measure_Num][2]=LRSRR_Input[k][2];
        | Measure_Data[Measure_Num][3]=LRSRR_Input[k][3];
        | Measure_Num++;
        | }
    (junction 1367) -> (junction 1368)
    (junction 1353) -> (junction 1352)
    (junction 1368) -> (junction 320) : {
        | k=0;
        | }
    (junction 320) -> (junction 1384) [order 1] : [DataSource==4]
    (junction 1384) -> (junction 1372) [order 1] : [k<10]
    (junction 1372) -> (junction 1370) [order 1] : [RRSRR_Input[k][0] !=0]
    (junction 1371) -> (junction 1384) : {
        | k++;
        | }
    (junction 320) -> (junction 325) [order 2]
    (junction 1384) -> (junction 1381) [order 2]
    (junction 1372) -> (junction 1371) [order 2]
    (junction 1370) -> (junction 1378) : {
        | Measure_Data[Measure_Num][0]=RRSRR_Input[k][0];
        | Measure_Data[Measure_Num][1]=RRSRR_Input[k][1];
        | Measure_Data[Measure_Num][2]=RRSRR_Input[k][2];
        | Measure_Data[Measure_Num][3]=RRSRR_Input[k][3];
        | Measure_Num++;
        | }
    (junction 1381) -> (junction 325)
    (junction 1378) -> (junction 1371)
    (junction 325) -> (junction 326) : {
        | k=0;
        | }
  state Possible_Cal [function]
    state Gtj_Cal [function]
      (default) -> (junction 412)
      (junction 412) -> (junction 413) [order 1] : [t<Num_Trg]
      (junction 413) -> (junction 414) [order 1] : [j<Measure_Num]
      (junction 415) -> (junction 412) : {
          | t++;
          | j=0;
          | }
      (junction 416) -> (junction 413) : {
          | j++;
          | }
      (junction 414) -> (junction 416) : {
          | Gtj[t][j]=G_cal(FusDataInternal[t][1],FusDataInternal[t][3],Measure_Data[j][1],Measure_Data[j][2],FusDataInternal[t][7],...
          | FusDataInternal[t][8],FusDataInternal[t][9],FusDataInternal[t][10],FusDataInternal[t][11],FusDataInternal[t][12],FusDataInternal[t][13],...
          | FusDataInternal[t][14],FusDataInternal[t][15],FusDataInternal[t][16],FusDataInternal[t][17],FusDataInternal[t][18],FusDataInternal[t][19],...
          | FusDataInternal[t][20],FusDataInternal[t][21],FusDataInternal[t][22],1.5,0,0,1.5);
          | %Assume that the radar variance is 1.5 and 1.5
          | }
      (junction 412) -> (junction 417) [order 2] : {
          | t=0;
          | j=0;
          | }
      (junction 413) -> (junction 415) [order 2]
    state Gsum_Cal [function]
      (default) -> (junction 433)
      (junction 433) -> (junction 447) [order 1] : [t<Num_Trg]
      (junction 447) -> (junction 449) [order 1] : [j<Measure_Num]
      (junction 451) -> (junction 433) : {
          | t++;
          | j=0;
          | }
      (junction 454) -> (junction 447) : {
          | j++;
          | }
      (junction 433) -> (junction 438) [order 2] : {
          | t=0;
          | j=0;
          | }
      (junction 447) -> (junction 451) [order 2]
      (junction 449) -> (junction 454) : {
          | Gtsum[t]=Gtsum[t]+Gtj[t][j];
          | }
      (junction 438) -> (junction 467) [order 1] : [j<Measure_Num]
      (junction 467) -> (junction 464) [order 1] : [t<Num_Trg]
      (junction 465) -> (junction 438) : {
          | j++;
          | t=0;
          | }
      (junction 466) -> (junction 467) : {
          | t++;
          | }
      (junction 438) -> (junction 468) [order 2] : {
          | t=0;
          | j=0;
          | }
      (junction 467) -> (junction 465) [order 2]
      (junction 464) -> (junction 466) : {
          | Gsumj[j]=Gsumj[j]+Gtj[t][j];
          | }
    state Ptj_Cal [function]
      (default) -> (junction 506)
      (junction 506) -> (junction 510) [order 1] : [t<Num_Trg]
      (junction 510) -> (junction 512) [order 1] : [j<Measure_Num]
      (junction 505) -> (junction 506) : {
          | t++;
          | j=0;
          | }
      (junction 502) -> (junction 510) : {
          | j++;
          | }
      (junction 506) -> (junction 514) [order 2] : {
          | t=0;
          | j=0;
          | }
      (junction 510) -> (junction 505) [order 2]
      (junction 512) -> (junction 502) : {
          | Ptj[t][j]=Gtj[t][j]/(Gtsum[t]+Gsumj[j]-Gtj[t][j]);
          | %calculate track t with all tracklet possible
          | }
      (junction 514) -> (junction 518)
    state Pt0_Cal [function]
      (default) -> (junction 523)
      (junction 523) -> (junction 524) [order 1] : [t<Num_Trg]
      (junction 524) -> (junction 525) [order 1] : [j<Measure_Num]
      (junction 527) -> (junction 523) : {
          | t++;
          | j=0;
          | }
      (junction 528) -> (junction 524) : {
          | j++;
          | }
      (junction 523) -> (junction 529) [order 2] : {
          | t=0;
          | j=0;
          | }
      (junction 524) -> (junction 527) [order 2]
      (junction 525) -> (junction 528) : {
          | Ptsum[t]=Ptsum[t]+Ptj[t][j];
          | %calculate sum of  track t with all tracklet possible
          | }
      (junction 529) -> (junction 550) [order 1] : [j<Measure_Num]
      (junction 550) -> (junction 545) [order 1] : [t<Num_Trg]
      (junction 544) -> (junction 529) : {
          | j++;
          | t=0;
          | }
      (junction 546) -> (junction 550) : {
          | t++;
          | }
      (junction 529) -> (junction 551) [order 2] : {
          | t=0;
          | j=0;
          | }
      (junction 550) -> (junction 544) [order 2]
      (junction 545) -> (junction 546) : {
          | Psumj[t]=Psumj[t]+Ptj[t][j];
          | %calculate sum of  tracklet j with all tracker possible
          | }
    (default) -> (junction 427)
    (junction 427) -> (junction 428) : {
        | Gtj_Cal();
        | Gsum_Cal();
        | Ptj_Cal();
        | Pt0_Cal();
        | }
    (junction 428) -> (junction 515)
  state Tracker_Manager [function]
    state FusTrackManage [function]
      state ExistScoreCal [function]
        state OutLFSRRFOV= OutLFSRRFOV [function]
          (default) -> (junction 1394)
          (junction 1394) -> (junction 1396) [order 1] : [(FusDataInternal_temp[t][3]-0.5*1.9-(-0.2679)*FusDataInternal_temp[t][1]>0) && ...
              | (FusDataInternal_temp[t][3]-0.5*1.9-(-1)*FusDataInternal_temp[t][1]>0)]
          (junction 1394) -> (junction 1399) [order 2] : {
              | OutLFSRRFOV=1;
              | }
          (junction 1396) -> (junction 1400) : {
              | OutLFSRRFOV=0;
              | }
          (junction 1400) -> (junction 1399)
          (junction 1399) -> (junction 1401)
        state OutRFSRRFOV= OutRFSRRFOV [function]
          (default) -> (junction 1423)
          (junction 1423) -> (junction 1424) [order 1] : [(FusDataInternal_temp[t][3]+0.5*1.9-(0.2679)*FusDataInternal_temp[t][1]<0) && ...
              | (FusDataInternal_temp[t][3]+0.5*1.9-(1)*FusDataInternal_temp[t][1]<0)]
          (junction 1423) -> (junction 1425) [order 2] : {
              | OutRFSRRFOV=1;
              | }
          (junction 1424) -> (junction 1426) : {
              | OutRFSRRFOV=0;
              | }
          (junction 1426) -> (junction 1425)
          (junction 1425) -> (junction 1427)
        state OutLRSRRFOV= OutLRSRRFOV [function]
          (default) -> (junction 1444)
          (junction 1444) -> (junction 1445) [order 1] : [(FusDataInternal_temp[t][3]-0.5*1.9-(0.2679)*(FusDataInternal_temp[t][1]+5.2)>0) && ...
              | (FusDataInternal_temp[t][3]-0.5*1.9-(1)*(FusDataInternal_temp[t][1]+5.2)>0)]
          (junction 1444) -> (junction 1446) [order 2] : {
              | OutLRSRRFOV=1;
              | }
          (junction 1445) -> (junction 1447) : {
              | OutLRSRRFOV=0;
              | }
          (junction 1447) -> (junction 1446)
          (junction 1446) -> (junction 1448)
        state OutRRSRRFOV= OutRRSRRFOV [function]
          (default) -> (junction 1468)
          (junction 1468) -> (junction 1469) [order 1] : [(FusDataInternal_temp[t][3]+0.5*1.9-(-0.2679)*(FusDataInternal_temp[t][1]+5.2)<0) && ...
              | (FusDataInternal_temp[t][3]+0.5*1.9-(-1)*(FusDataInternal_temp[t][1]+5.2)<0)]
          (junction 1468) -> (junction 1470) [order 2] : {
              | OutRRSRRFOV=1;
              | }
          (junction 1469) -> (junction 1471) : {
              | OutRRSRRFOV=0;
              | }
          (junction 1471) -> (junction 1470)
          (junction 1470) -> (junction 1472)
        (default) -> (junction 974)
        (junction 974) -> (junction 973) [order 1] : [UpdateTrackFlag[t]==1]
        (junction 974) -> (junction 1385) [order 2]
        (junction 973) -> (junction 983) : {
            | FusDataInternal_temp[t][23]=FusDataInternal_temp[t][23]+4;
            | }
        (junction 1385) -> (junction 1387) [order 1] : [(DataSource==1) && (OutLFSRRFOV()==1)]%Source is LFSRR and out of FOV
        (junction 1385) -> (junction 1413) [order 2]
        (junction 1387) -> (junction 1389)
        (junction 1413) -> (junction 1415) [order 1] : [(DataSource==2) && (OutRFSRRFOV()==1)]%Source is RFSRR and out of FOV
        (junction 1413) -> (junction 1436) [order 2]
        (junction 1415) -> (junction 1417)
        (junction 983) -> (junction 984) [order 1] : [FusDataInternal_temp[t][23]>18]
        (junction 983) -> (junction 988) [order 2]
        (junction 984) -> (junction 989) : {
            | FusDataInternal_temp[t][23]=18;
            | }
        (junction 1436) -> (junction 1437) [order 1] : [(DataSource==3) && (OutLRSRRFOV()==1)]%Source is LRSRR and out of FOV
        (junction 1436) -> (junction 1456) [order 2]
        (junction 1437) -> (junction 1438)
        (junction 1456) -> (junction 1458) [order 1] : [(DataSource==4) && (OutRRSRRFOV()==1)]%Source is RRSRR and out of FOV
        (junction 1456) -> (junction 1462) [order 2] : {
            | FusDataInternal_temp[t][23]=FusDataInternal_temp[t][23]-3;
            | }
        (junction 1458) -> (junction 1459)
        (junction 1459) -> (junction 1462)
        (junction 1438) -> (junction 1459)
        (junction 1417) -> (junction 1438)
        (junction 1389) -> (junction 1417)
        (junction 988) -> (junction 1389)
        (junction 989) -> (junction 988)
        (junction 1462) -> (junction 985)
      state OutputTrack [function]
        (default) -> (junction 1187)
        (junction 1188) -> (junction 1189) [order 1] : [FusDataInternal_temp[t][23]<15]
        (junction 1187) -> (junction 1188) [order 1] : [FusDataInternal_temp[t][24]==0]%Not a confirmed track
        (junction 1189) -> (junction 1199) : {
            | TrackCounter++;
            | }
        (junction 1187) -> (junction 1190) [order 2]
        (junction 1188) -> (junction 1191) [order 2] : {
            | FusDataInternal_temp[t][24]=1;
            | %New confirmed track
            | }
        (junction 1191) -> (junction 1190)
        (junction 1190) -> (junction 1192) : {
            | SideFusOut[Num_Out][0]=FusDataInternal_temp[t][0];%ID
            | SideFusOut[Num_Out][1]=FusDataInternal_temp[t][1];%Range X
            | SideFusOut[Num_Out][2]=FusDataInternal_temp[t][3];%Range Y
            | SideFusOut[Num_Out][3]=FusDataInternal_temp[t][5];% Move Info
            | %Select outputs signals from Internal to output
            | TrackCounter++;Num_Out++;
            | }
        (junction 1192) -> (junction 1193) [order 1] : [FusDataInternal_temp[t][23]<=15]
        (junction 1193) -> (junction 1194) [order 1] : [FusDataInternal_temp[t][23]<=9]
        (junction 1192) -> (junction 1195) [order 2] : {
            | %FusDataOut[Num_Out-1][6]=3;
            | %High confidence
            | }
        (junction 1193) -> (junction 1196) [order 2] : {
            | %FusDataOut[Num_Out-1][6]=2;
            | %Speculative
            | }
        (junction 1194) -> (junction 1197) : {
            | %FusDataOut[Num_Out-1][6]=1;
            | %High Speculative
            | }
        (junction 1196) -> (junction 1195)
        (junction 1197) -> (junction 1196)
        (junction 1195) -> (junction 1198)
        (junction 1199) -> (junction 1198)
        (junction 1198) -> (junction 1200)
      state Del_InternalTrack [function]
        (default) -> (junction 1220) : {
            | IDUsedFlag[FusDataInternal_temp[t][0]]=0;%Reflash ID Used Flag
            | }
        (junction 1220) -> (junction 1221) [order 1] : [c<24]
        (junction 1222) -> (junction 1220) : {c++;}
        (junction 1220) -> (junction 1223) [order 2] : {
            | c=0;
            | TrackCounter++;
            | }
        (junction 1221) -> (junction 1222) : {
            | FusDataInternal_temp[t][c]=0;
            | }
      (default) -> (junction 959)
      (junction 959) -> (junction 960) : {
          | ExistScoreCal();
          | }
      (junction 960) -> (junction 961) [order 1] : [FusDataInternal_temp[t][23]>=0]%Marks >=0
      (junction 960) -> (junction 962) [order 2] : {
          | Del_InternalTrack();
          | }
      (junction 961) -> (junction 963) : {
          | OutputTrack();
          | }
      (junction 963) -> (junction 962)
      (junction 962) -> (junction 964)
    (default) -> (junction 829)
    (junction 829) -> (junction 830) [order 1] : [t<Num_Trg]
    (junction 832) -> (junction 829) : {
        | t++;
        | }
    (junction 829) -> (junction 831) [order 2] : {
        | t=0;
        | }
    (junction 830) -> (junction 832) : {
        | FusTrackManage();
        | }
  state DataSet [parallel]
    settings: executionOrder=1
    state A
    (default) -> A
    A -> (junction 1232)
    (junction 1232) -> (junction 1233) [order 1] : LFSRR%Left Front SRR_Update
    (junction 1232) -> (junction 1234) [order 2]
    (junction 1233) -> (junction 1241) : {
        | Set_Source(1);
        | Set_Time(LFSRR_RxTm);
        | }
    (junction 1234) -> (junction 1235) [order 1] : RFSRR%Right Front SRR Update
    (junction 1234) -> (junction 1236) [order 2]
    (junction 1235) -> (junction 1240) : {
        | Set_Source(2);
        | Set_Time(RFSRR_RxTm);
        | }
    (junction 1236) -> (junction 1237) [order 1] : LRSRR%Left Rear SRR_Update
    (junction 1236) -> (junction 1238) [order 2]
    (junction 1237) -> (junction 1239) : {
        | Set_Source(3);
        | Set_Time(LRSRR_RxTm);
        | }
    (junction 1238) -> (junction 1262) [order 1] : RRSRR%Right Rear SRR_Update
    (junction 1238) -> (junction 1242) [order 2]
    (junction 1262) -> (junction 1264) : {
        | Set_Source(4);
        | Set_Time(RRSRR_RxTm);
        | }
    (junction 1264) -> (junction 1242)
    (junction 1239) -> (junction 1264)
    (junction 1240) -> (junction 1239)
    (junction 1241) -> (junction 1240)
    (junction 1242) -> DataSet
  state Fusion_Main [parallel]
    settings: executionOrder=2
    state B
    (default) -> B
    B -> (junction 202)
    (junction 202) -> (junction 1311) : {
        | FusDataIni();
        | FusTrackPredict();
        | Measurement_Gen();
        | Possible_Cal();
        | Tracker_Update();
        | Tracker_Manager();
        | Tracker_Initial();
        | }
    (junction 1311) -> (junction 203) : {
        | LastCalTime=Sensor_sampleTime;
        | Num_Trg=TrackCounter;
        | }
    (junction 203) -> (junction 1292) [order 1] : [GlobalFusTrgCount>3]
    (junction 203) -> (junction 1296) [order 2] : {
        | GlobalFusTrgCount++;
        | }
    (junction 1292) -> (junction 3562) : {
        | GlobalFusTrgCount=0;
        | }
    (junction 3562) -> (junction 3563) [order 1] : [Global_Fus_Event==1]
    (junction 3562) -> (junction 1294) [order 2] : {
        | Global_Fus_Event=1;
        | }
    (junction 3563) -> (junction 3565) : {
        | Global_Fus_Event=0;
        | }
    (junction 1294) -> (junction 1296)
    (junction 3565) -> (junction 1294)
    (junction 1296) -> Fusion_Main
  data: xt function_input; yt function_input; xj function_input; yj function_input; P11 function_input; P12 function_input; P13 function_input; P14 function_input; P21 function_input; P22 function_input; P23 function_input; P24 function_input; P31 function_input; P32 function_input; P33 function_input; P34 function_input; P41 function_input; P42 function_input; P43 function_input; P44 function_input; R11 function_input; Gtj function_output; R12 function_input; R21 function_input; R22 function_input; data function_input double; Pre_x function_input; Pre_vx function_input; Pre_y function_input; Pre_vy function_input; pre_p11 function_input; pre_p12 function_input; pre_p13 function_input; pre_p14 function_input; pre_p21 function_input; pre_p22 function_input; pre_p23 function_input; pre_p24 function_input; pre_p31 function_input; pre_p32 function_input; pre_p33 function_input; pre_p34 function_input; pre_p41 function_input; pre_p42 function_input; pre_p43 function_input; pre_p44 function_input; mk function_input; RangeX function_output; VelX function_output; RangeY function_output; VelY function_output; P11 function_output; P12 function_output; P13 function_output; P14 function_output; P21 function_output; P22 function_output; P23 function_output; P24 function_output; P31 function_output; P32 function_output; P33 function_output; P34 function_output; P41 function_output; P42 function_output; P43 function_output; P44 function_output; m00 function_input; m01 function_input; m2 function_input; m10 function_input; m11 function_input; m12 function_input; m20 function_input; m21 function_input; m22 function_input; Pt0 function_input; data function_input double; Pre_x function_input; Pre_vx function_input; Pre_y function_input; Pre_vy function_input; deltaT function_input; pre_p11 function_input; pre_p12 function_input; pre_p13 function_input; pre_p14 function_input; pre_p21 function_input; pre_p22 function_input; pre_p23 function_input; pre_p24 function_input; pre_p31 function_input; pre_p32 function_input; pre_p33 function_input; pre_p34 function_input; pre_p41 function_input; pre_p42 function_input; pre_p43 function_input; pre_p44 function_input; RangeX function_output; VelX function_output; RangeY function_output; VelY function_output; P11 function_output; P12 function_output; P13 function_output; P14 function_output; P21 function_output; P22 function_output; P23 function_output; P24 function_output; P31 function_output; P32 function_output; P33 function_output; P34 function_output; P41 function_output; P42 function_output; P43 function_output; P44 function_output; x_t function_input; y_t function_input; x_m function_input; y_m function_input; vx_max function_input; vx_min function_input; vy_max function_input; vy_min function_input; Rxx function_input; Ryy function_input; AssociationFlag function_output; threshod function_input; ts function_input; x1 function_input; y1 function_input; x2 function_input; y2 function_input; xm function_input; ym function_input; relative_degree function_output; ini_x function_input double; ini_y function_input double; h temporary double =0; OutLFSRRFOV function_output double; h temporary double =0; OutRFSRRFOV function_output double; h temporary double =0; OutLRSRRFOV function_output double; h temporary double =0; OutRRSRRFOV function_output double; LFSRR_Input input double size=[10 4]; LFSRR_RxTm input double; RFSRR_Input input double size=[10 4]; RFSRR_RxTm input double; LRSRR_Input input double size=[10 4]; FusDataInternal local double size=[40 25]; Gtj local double size=[40 40]; Ptj local double size=[40 40]; deltaT local double size=1 =0; k local double size=1 =0; Measure_Data local double size=[40 5] =0; Measure_Num local double size=1 =0; Tracker_Num local double size=1 =0; FusDataInternal_temp local double size=[40 25]; n local double size=1 =0; t local double size=1 =0; j local double size=1 =0; Gtsum local double size=40; Gsumj local double size=40; Pt0 local double size=40; Ptsum local double size=40; Psumj local double size=40; P_Bulb local double size=[40 4]; P_Bulbtemp0 local double size=1 =0; P_Bulbtemp1 local double size=1 =0; P_Bulbtemp2 local double size=1 =0; SelectMea local double size=[3 3] =0; P_Bulbtemp3 local double size=1 =0; UpdateTrackFlag local double size=40 =0; LRSRR_RxTm input double; RRSRR_Input input double size=[10 4]; RRSRR_RxTm input double; SideFusOut output double size=[40 4]; GlobalFusTrgCount local double =0; Sensor_sampleTime local double; LastCalTime local double size=1 =240; Num_Trg local double size=1 =0; TrackCounter local double size=1 =0; c local double size=1 =0; Num_Out local double size=1 =0; Num_Returns local double size=1 =0; Returns local double size=[10 3] =0; Ini_Tracker_LFSRR local double size=[100 14] =0; Ini_Tracker_RFSRR local double size=[100 14] =0; Ini_Tracker_LRSRR local double size=[100 14] =0; Ini_Tracker_RRSRR local double size=[100 14] =0; Num_Ini_Tracker_RFSRR local double size=1 =0; Num_Ini_Tracker_LFSRR local double size=1 =0; Num_Ini_Tracker_LRSRR local double size=1 =0; Num_Ini_Tracker_RRSRR local double size=1 =0; AssoFlgtm local double size=10 =0; Ini_Tracker_LFSRR_New local double size=[100 14] =0; Ini_Tracker_LRSRR_New local double size=[100 14] =0; Ini_Tracker_RFSRR_New local double size=[100 14] =0; Ini_Tracker_RRSRR_New local double size=[100 14] =0; Num_Ini_Tracker_LFSRR_New local double size=1 =0; Num_Ini_Tracker_LRSRR_New local double size=1 =0; Num_Ini_Tracker_RFSRR_New local double size=1 =0; Num_Ini_Tracker_RRSRR_New local double size=1 =0; RelDeg local double size=1 =0; x_3_predict local double size=1 =0; x_5_predict local double size=1 =0; x_4_predict local double size=1 =0; y_4_predict local double size=1 =0; y_3_predict local double size=1 =0; y_5_predict local double size=1 =0; Min_Distance_IniTrack local double size=1 =0; RelativeDist local double size=1 =0; Ini_Tracker_UpdateFlg local double size=1 =0; Updatereturn local double size=1 =0; LastFusID local double size=1 =0; IDUsedFlag local double size=127; LoopError local double size=1 =0; DataSource local double size=1 =0; LoopFlg local double size=1 =0; mk local double size=1 =0; OneMeasureFlg local double size=10 =0; Poss_Threshold_unused constant double size=1 =0.06; Poss_Threshold_used constant double size=1 =0.15; Group_Data local double size=[10 2]; Group_Num local double size=1 =0; Group_X local double size=1 =0; Group_Y local double size=1 =0; Global_Fus_Event output double size=1 =0
  events: LFSRR input FUNCTION_CALL_EVENT; RFSRR input FUNCTION_CALL_EVENT; LRSRR input FUNCTION_CALL_EVENT; RRSRR input FUNCTION_CALL_EVENT
